simulink model "LoadFlow116BusNetwork_original"  (R2024a)
settings: Solver=FixedStepDiscrete  StartTime=0.0  StopTime=4.5  FixedStep=75e-6  RelTol=1e-3  EnableMultiTasking=on
undefined symbols (not defined in the file or in its folder): D1, D11, Delta
libraries: spsSeriesRLCBranchLib x164, spsLoadFlowBusLib x116, spsDistributedParametersLineLib x79, spsThreePhaseSeriesRLCLoadLib x60, spsThreePhaseTransformerTwoWindingsLib x52, spsThreePhaseParallelRLCLoadLib x44, spsThreePhaseVIMeasurementLib x44, spsSynchronousMachinepuStandardLib x28, spsExcitationSystemLib x28, spsHydraulicTurbineandGovernorLib x28, spsGenericPowerSystemStabilizerLib x28, spsMultiBandPowerSystemStabilizerLib x28
(part 1 of 15)
settings Model: Creator=The MathWorks, Inc.  LastModifiedBy=dilu2
settings SolverCC: AlgebraicLoopSolver=TrustRegion
settings DataIOCC: SaveFormat=StructureWithTime  SaveOutput=off  SignalLogging=off  DSMLogging=off  SaveTime=off  ReturnWorkspaceOutputs=off
settings OptimizationCC: ExpressionDepthLimit=2147483647  LifeSpan=inf
settings DebuggingCC: UnderspecifiedInitializationDetection=Classic  MergeDetectMultiDrivingBlocksExec=none  SolverPrmCheckMsg=warning  FcnCallInpInsideContextMsg=warning  UnconnectedInputMsg=warning  UnconnectedOutputMsg=warning  UnconnectedLineMsg=warning  StateNameClashWarn=warning  SFUnexpectedBacktrackingDiag=warning  SFNoUnconditionalDefaultTransitionDiag=warning  SFExecutionAtInitializationDiag=none  ArithmeticOperatorsInVariantConditions=warning
settings HardwareCC: ProdBitPerPointer=32  ProdBitPerSizeT=32  ProdBitPerPtrDiffT=32  ProdLargestAtomicFloat=None  ProdIntDivRoundTo=Undefined  ProdEndianess=Unspecified  ProdWordSize=32  ProdHWDeviceType=32-bit Generic
settings ModelReferenceCC: EnableRefExpFcnMdlSchedulingChecks=on  PropagateSignalLabelsOutOfModel=off
settings SFSimCC: SimUseLocalCustomCode=off  CustomCodeUndefinedFunction=UseInterfaceOnly
settings RTWCC: RTWUseLocalCustomCode=off  GPUComputeCapability=3.5
settings CodeAppCC: StateflowObjectComments=on
settings GRTTargetCC: TargetLangStandard=C89/C90 (ANSI)  CombineOutputUpdateFcns=off  GRTInterface=on
settings ConfigComp: CovMetricSettings=dw  CovSaveCumulativeToWorkspaceVar=on  CovSaveSingleToWorkspaceVar=on  CovExternalEMLEnable=off  CovSFcnEnable=off
settings SimscapeCC: SimscapeNormalizeSystem=off

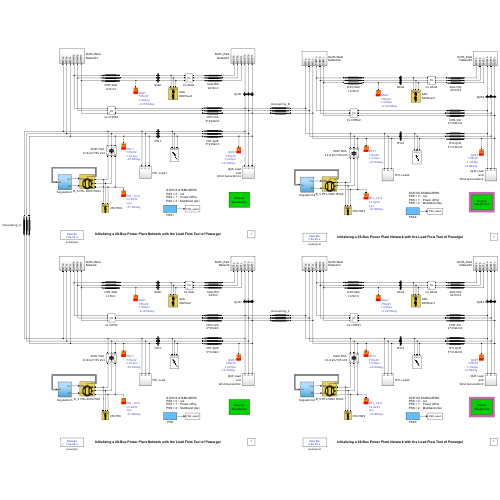
[thumbnail: Simulink's stored preview of the top-level diagram]
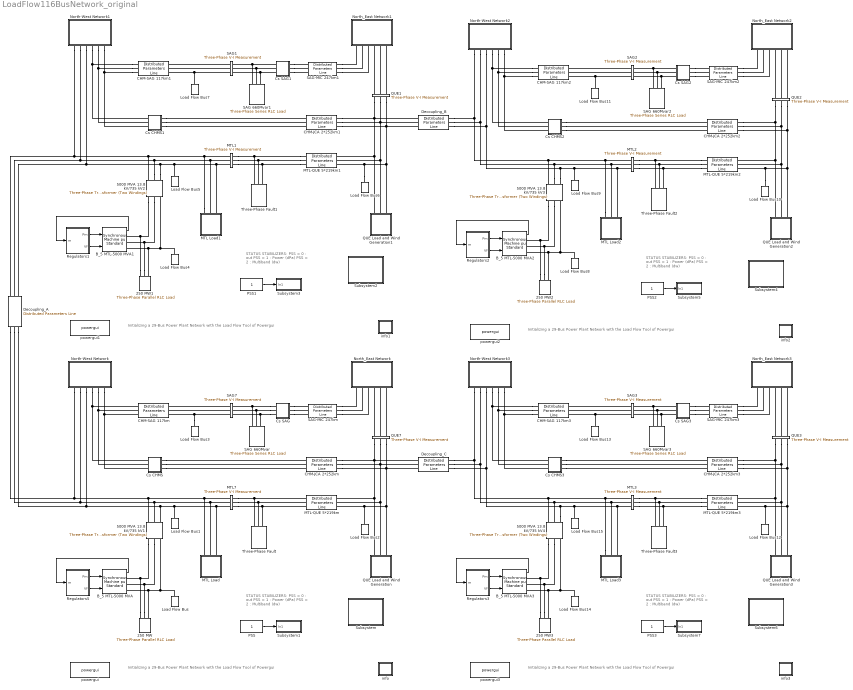
== system LoadFlow116BusNetwork_original ==
  note: Initializing a 29-Bus Power Plant Network with the Load Flow Tool of Powergui
  note: STATUS STABILIZERS:
      | PSS = 0 :  out
      | PSS = 1 :  Power (dPa)
      | PSS = 2 :  Multiband (dw)
  note: STATUS STABILIZERS:
      | PSS = 0 :  out
      | PSS = 1 :  Power (dPa)
      | PSS = 2 :  Multiband (dw)
  note: Initializing a 29-Bus Power Plant Network with the Load Flow Tool of Powergui
  note: Initializing a 29-Bus Power Plant Network with the Load Flow Tool of Powergui
  note: STATUS STABILIZERS:
      | PSS = 0 :  out
      | PSS = 1 :  Power (dPa)
      | PSS = 2 :  Multiband (dw)
  note: STATUS STABILIZERS:
      | PSS = 0 :  out
      | PSS = 1 :  Power (dPa)
      | PSS = 2 :  Multiband (dw)
  note: Initializing a 29-Bus Power Plant Network with the Load Flow Tool of Powergui
  250 MW{,1..3} (4 alike) : spsThreePhaseParallelRLCLoadLib/Three-Phase Parallel RLC Load  LConnTagsString=A|B|C  Configuration=Y (grounded)  NominalVoltage=(13800)*1  Vabc=[1e3 1e3 1e3]  Vabcp=[1e3 1e3 1e3]  NominalFrequency=60  UnbalancedPower=off  ActivePower=250000000  InductivePower=0  CapacitivePower=0  Pabc=[10e3 9e3 11e3]  QLabc=[100 90 110]  QCabc=[100 90 110]  Pabcp=[10e3 9e3 11e3]  QLabcp=[100 90 110]  QCabcp=[100 90 110]  Measurements=None  LoadType=constant PQ
  5000 MVA 13.8 kV/735 kV{1..4} (4 alike) : spsThreePhaseTransformerTwoWindingsLib/Three-Phase Transformer (Two Windings)  Winding1Connection=Delta (D1)  Winding2Connection=Yg  CoreType=Three single-phase transformers  SetSaturation=off  Hysteresis=off  DataFile='basic_model'  SetInitialFlux=off  Measurements=None  UNITS=pu  NominalPower=[ 5000e6 60 ]  Winding1="[ 13.8e3 0.002  0.0]"  Winding2=[ 735e3 0.002 0.12]  Rm=500  Lm=500  L0=0.5  Saturation="[ 0,0  ;  0.005,1.2  ;  1.0,1.4 ]"  InitialFluxes=[ 0.8 , -0.8 , 0.7 ]  BreakLoop=off  DiscreteSolver=Trapezoidal iterative  DataType=off  TransfoNumber=0
  B_5 MTL-5000 MVA{,1..3} (4 alike) : spsSynchronousMachinepuStandardLib/Synchronous Machine pu Standard  PresetModel=No  MechanicalLoad=Mechanical power Pm  ShowDetailedParameters=on  RotorType=Salient-pole  Units=per unit standard parameters  MeasurementBus=off  NominalParameters="[5000E6  13800   60 ]"  Reactances1=[ 31 32 33 34 35 36 37 ]  Reactances2=[ 1.305, 0.296, 0.252, 0.474, 0.243, 0.18 ]  dAxisTimeConstants=Short-circuit  qAxisTimeConstants=Open-circuit  TimeConstants1=[]  TimeConstants2=[]  TimeConstants3=[]  TimeConstants4=[]  TimeConstants5=[ 1.01, 0.053, 0.1 ]  TimeConstants6=[]  TimeConstants7=[]  TimeConstants8=[]  StatorResistance=2.8544e-3  Mechanical="[ 3.7 0  32]"  PolePairs=32  InitialConditions=[0 -113.876 0.904539 0.904539 0.904539 -42.1129 -162.113 77.8871 1.28555]  SetSaturation=off  Saturation=[0.6404,0.7127,0.8441,0.9214,0.9956,1.082,1.19,1.316,1.457;0.7,0.7698,0.8872,0.9466,0.9969,1.046,1.1,1.151,1.201]  LoadFlowParameters=[1 4000000000 0 0 0]  TsPowergui=0  TsBlock=-1  IterativeModel=Trapezoidal non iterative  IterativeDiscreteModel=Trapezoidal non iterative  BusType=PV  Pref=4500000000  Qref=0  Qmin=-Inf  Qmax=Inf  PLF=0  QLF=0
  CHM-JCA 2*252km : spsDistributedParametersLineLib/Distributed Parameters Line  Phases=3  Length=252  Frequency=60  Resistance="[0.01273  0.3864]/2"  Inductance="[0.9337e-3  4.1264e-3]/2"  Capacitance=[12.74e-9 7.751e-9]*2  x1=[-0.0015 2.79983584355551e-08 40957.0521348616 -638802.206166497;-0.001425 2.7893105015594e-08 58999.9677158828 -637388.990068573;-0.00135 2.77655542742622e-08 76995.7196254415 -635466.254964366;-0.001275 2.76158081736708e-08 94929.9223348058 -633035.537858901;-0.0012 2.74439864185614e-08 112788.239516732 -630098.78183024;-0.001125 2.72502263606161e-08 130556.395505707 -626658.334476219;-0.00105 2.70346828886605e-08 148220.186709694 -622716.946037811;-0.000975 2.67975283048483e-08 165765.49296427 -618277.767200629;-0.0009 2.65389521869251e-08 183178.288820068 -613344.346576314;-0.000825 2.62591612366833e-08 200444.654754505 -607920.62786583;-0.00075 2.59583791147275e-08 217550.788298837 -602010.946706926;-0.000675 2.56368462616839e-08 234483.015071642 -595620.027208302;-0.0006 2.52948197059956e-08 251227.799709909 -588752.978173219;-0.000525 2.49325728584581e-08 267771.756689002 -581415.289015608;-0.00045 2.45503952936587e-08 284101.661022843 -573612.825371909;-0.000375 2.41485925184951e-08 300204.458835764 -565351.824412179;-0.0003 2.37274857279582e-08 316067.277797573 -556638.889854187;-0.000225 2.3287411548373e-08 331677.437413503 -547480.986684506;-0.00015 2.28287217683054e-08 347022.459160799 -537885.435590809;-7.5e-05 2.23517830573473e-08 362090.076463864 -527859.907109824]  x2=[-0.0015 1.96439398291852e-08 -210407.400599635 -626129.029139422;-0.001425 1.95042039382265e-08 -192622.277099833 -631827.111409279;-0.00135 1.93488766850639e-08 -174683.174298938 -637020.120753555;-0.001275 1.91780822359271e-08 -156604.43244125 -641703.905960035;-0.0012 1.89919571212853e-08 -138400.503396396 -645874.72288249;-0.001125 1.87906501267075e-08 -120085.939106726 -649529.237433687;-0.00105 1.85743221739249e-08 -101675.379954711 -652664.52825061;-0.000975 1.83431461921932e-08 -83183.5430596452 -655278.089029752;-0.0009 1.8097306980055e-08 -64625.2105130086 -657367.830530614;-0.000825 1.7837001057615e-08 -46015.2175618868 -658932.082245816;-0.00075 1.75624365094449e-08 -27368.4407499025 -659969.593736469;-0.000675 1.72738328182434e-08 -8699.7860251338 -660479.535631762;-0.0006 1.69714206893854e-08 9975.82317547212 -660461.500291947;-0.000525 1.66554418664999e-08 28643.4578556668 -659915.502134199;-0.00045 1.6326148938223e-08 47288.1953939113 -658841.97762109;-0.000375 1.59838051362834e-08 65895.1314722915 -657241.784911691;-0.0003 1.56286841250783e-08 84449.3919908021 -655116.203175571;-0.000225 1.52610697829104e-08 102936.144957474 -652466.931570246;-0.00015 1.48812559750603e-08 121340.612344843 -649296.087882902;-7.5e-05 1.44895463188746e-08 139648.081903277 -645606.206837468]  x3=[-0.0015 6.74615242643494e-11 -389.356346677576 1012.15852814398;-0.001425 6.66063511630319e-11 -417.814729884147 1000.74710827411;-0.00135 6.56979339637061e-11 -445.939118388429 988.535706477818;-0.001275 6.47369988411817e-11 -473.707029984568 975.534084362876;-0.0012 6.37243139522931e-11 -501.096267428898 961.752635227066;-0.001125 6.26606888218456e-11 -528.084936184076 947.202375749965;-0.00105 6.15469736954946e-11 -554.651461921238 931.894937186371;-0.000975 6.03840588600718e-11 -580.774607766193 915.842556068461;-0.0009 5.91728739319033e-11 -606.433491275848 899.058064424092;-0.000825 5.7914387113689e-11 -631.607601131322 881.554879519071;-0.00075 5.66096044205358e-11 -656.276813534371 863.346993131604;-0.000675 5.52595688757648e-11 -680.421408294053 844.44896036748;-0.0006 5.38653596771343e-11 -704.022084590741 824.875888024941;-0.000525 5.24280913341456e-11 -727.059976404907 804.643422518539;-0.00045 5.0948912777121e-11 -749.516667598325 783.767737371633;-0.000375 4.94290064387669e-11 -771.374206635655 762.26552028752;-0.0003 4.78695873089548e-11 -792.615120934621 740.153959809543;-0.000225 4.62719019634771e-11 -813.22243083333 717.45073158083;-0.00015 4.46372275675538e-11 -833.179663163552 694.173984214655;-7.5e-05 4.29668708548854e-11 -852.470864419117 670.342324786718]  x4=[-0.0015 5.35912228760876e-11 -2387.01909458833 -10068.0123244672;-0.001425 5.47734177538654e-11 -2101.43699245865 -10131.4710131204;-0.00135 5.59118275995522e-11 -1814.17503375026 -10186.8307588624;-0.001275 5.70055423857356e-11 -1525.4628512777 -10234.0473079595;-0.0012 5.80536878135499e-11 -1235.5312371422 -10273.0829162248;-0.001125 5.90554260115772e-11 -944.611958239979 -10303.9063791903;-0.00105 6.00099562056291e-11 -652.937570991393 -10326.4930570513;-0.000975 6.09165153588735e-11 -360.741235438837 -10340.8248943632;-0.0009 6.17743787817938e-11 -68.2565288621972 -10346.8904344744;-0.000825 6.25828607114957e-11 224.282740939255 -10344.6848286851;-0.00075 6.33413148598947e-11 516.642722549241 -10334.2098401227;-0.000675 6.40491349303493e-11 808.589707871721 -10315.4738423328;-0.0006 6.47057551023253e-11 1099.89031895356 -10288.4918125854;-0.000525 6.53106504837036e-11 1390.31169454332 -10253.2853199022;-0.00045 6.58633375303718e-11 1679.62167623695 -10209.8825078148;-0.000375 6.63633744327611e-11 1967.58899406166 -10158.3180718671;-0.0003 6.68103614690224e-11 2253.98345134964 -10098.6332318802;-0.000225 6.72039413245583e-11 2538.57610875372 -10030.875699002;-0.00015 6.75437993776541e-11 2821.13946725797 -9955.09963756763;-7.5e-05 6.78296639509821e-11 3101.44765003698 -9871.36562180108]  x5=0.00142516474882927  V1=ones(3,3)  V2=ones(3,3)  I1=ones(3,3)  I2=ones(3,3)  nHarmo=1  Measurements=None  Decoupling=off  VsMag0=[ 1 1 1]  VrMag0=[ 1 1 1]  VsAngle0=[0 -120 120]  VrAngle0=[0 -120 120]  IsMag0=[ 1 1 1]  IrMag0=[ 1 1 1]  IsAngle0=[0 -120 120]  IrAngle0=[0 -120 120]
      settings: AttributesFormatString=\n  LibrarySourceBlock=sps_lib/Power Grid Elements/Distributed Parameters Line
  CHM-JCA 2*252km1 : spsDistributedParametersLineLib/Distributed Parameters Line  Phases=3  Length=252  Frequency=60  Resistance="[0.01273  0.3864]/2"  Inductance="[0.9337e-3  4.1264e-3]/2"  Capacitance=[12.74e-9 7.751e-9]*2  x1=[-0.0015 7.55859688120085e-09 40957.0521347763 -638802.206166561;-0.001425 7.87146395364578e-09 58999.9677157988 -637388.990068633;-0.00135 8.17803869824361e-09 76995.7196253592 -635466.254964424;-0.001275 8.47807604383424e-09 94929.922334725 -633035.537858955;-0.0012 8.77133614515435e-09 112788.239516653 -630098.781830291;-0.001125 9.05758457456597e-09 130556.395505629 -626658.334476266;-0.00105 9.33659250945436e-09 148220.186709618 -622716.946037854;-0.000975 9.60813691514536e-09 165765.492964196 -618277.767200669;-0.0009 9.87200072319581e-09 183178.288819996 -613344.346576351;-0.000825 1.01279730049148e-08 200444.654754435 -607920.627865863;-0.00075 1.03758491399769e-08 217550.788298769 -602010.946706956;-0.000675 1.06154309799923e-08 234483.015071576 -595620.027208328;-0.0006 1.08465270069038e-08 251227.799709845 -588752.978173242;-0.000525 1.10689524860834e-08 267771.75668894 -581415.289015627;-0.00045 1.12825296140063e-08 284101.661022783 -573612.825371925;-0.000375 1.14870876603843e-08 300204.458835706 -565351.824412191;-0.0003 1.16824631046448e-08 316067.277797518 -556638.889854195;-0.000225 1.18684997666472e-08 331677.43741345 -547480.98668451;-0.00015 1.20450489315303e-08 347022.459160749 -537885.43559081;-7.5e-05 1.2211969468593e-08 362090.076463816 -527859.907109821]  x2=[-0.0015 5.57833938393212e-09 -210407.400599694 -626129.029139484;-0.001425 5.75756020399417e-09 -192622.277099891 -631827.111409339;-0.00135 5.93217851852278e-09 -174683.174298994 -637020.120753612;-0.001275 6.10205474030905e-09 -156604.432441306 -641703.90596009;-0.0012 6.26705307290048e-09 -138400.503396451 -645874.722882543;-0.001125 6.42704161915457e-09 -120085.93910678 -649529.237433737;-0.00105 6.58189248667534e-09 -101675.379954764 -652664.528250658;-0.000975 6.73148189004859e-09 -83183.5430596976 -655278.089029798;-0.0009 6.87569024979407e-09 -64625.21051306 -657367.830530658;-0.000825 7.01440228795544e-09 -46015.2175619372 -658932.082245856;-0.00075 7.14750712025178e-09 -27368.4407499517 -659969.593736507;-0.000675 7.27489834471672e-09 -8699.78602518191 -660479.535631798;-0.0006 7.39647412675457e-09 9975.8231754252 -660461.50029198;-0.000525 7.51213728054534e-09 28643.4578556211 -659915.502134229;-0.00045 7.62179534673359e-09 47288.1953938668 -658841.977621118;-0.000375 7.72536066633905e-09 65895.1314722483 -657241.784911716;-0.0003 7.82275045082982e-09 84449.3919907603 -655116.203175593;-0.000225 7.91388684830229e-09 102936.144957434 -652466.931570265;-0.00015 7.99869700571475e-09 121340.612344804 -649296.087882919;-7.5e-05 8.07711312712502e-09 139648.08190324 -645606.206837482]  x3=[-0.0015 3.15277693640631e-11 -389.356346677657 1012.15852814422;-0.001425 3.20576641633681e-11 -417.814729884204 1000.74710827436;-0.00135 3.25619325564397e-11 -445.939118388461 988.535706478099;-0.001275 3.30401714388399e-11 -473.707029984576 975.534084363178;-0.0012 3.34919985137235e-11 -501.096267428882 961.752635227389;-0.001125 3.39170525974399e-11 -528.084936184035 947.202375750308;-0.00105 3.43149939082583e-11 -554.651461921173 931.894937186735;-0.000975 3.46855043379834e-11 -580.774607766104 915.842556068845;-0.0009 3.50282877062468e-11 -606.433491275735 899.058064424495;-0.000825 3.53430699972685e-11 -631.607601131185 881.554879519494;-0.00075 3.56295995789016e-11 -656.27681353421 863.346993132046;-0.000675 3.58876474037824e-11 -680.421408293868 844.448960367941;-0.0006 3.6117007192428e-11 -704.022084590533 824.87588802542;-0.000525 3.63174955981328e-11 -727.059976404675 804.643422519036;-0.00045 3.64889523535328e-11 -749.51666759807 783.767737372148;-0.000375 3.6631240398721e-11 -771.374206635377 762.265520288052;-0.0003 3.67442459908112e-11 -792.61512093432 740.153959810092;-0.000225 3.68278787948623e-11 -813.222430833007 717.450731581396;-0.00015 3.68820719560901e-11 -833.179663163206 694.173984215237;-7.5e-05 3.69067821533109e-11 -852.470864418749 670.342324787315]  x4=[-0.0015 -1.01395513576639e-11 -2387.01909458939 -10068.0123244686;-0.001425 -9.2349393761498e-12 -2101.43699245972 -10131.4710131218;-0.00135 -8.32294512539771e-12 -1814.17503375135 -10186.8307588638;-0.001275 -7.40429763965771e-12 -1525.4628512788 -10234.0473079608;-0.0012 -6.47973127167411e-12 -1235.53123714331 -10273.0829162261;-0.001125 -5.54998510565516e-12 -944.611958241099 -10303.9063791916;-0.00105 -4.61580236646036e-12 -652.937570992522 -10326.4930570526;-0.000975 -3.67792982547795e-12 -360.741235439974 -10340.8248943645;-0.0009 -2.73711720366728e-12 -68.2565288633418 -10346.8904344757;-0.000825 -1.79411657224329e-12 224.282740938104 -10344.6848286863;-0.00075 -8.49681751482354e-13 516.642722548085 -10334.2098401239;-0.000675 9.54322918701537e-14 808.589707870561 -10315.4738423339;-0.0006 1.0404700481087e-12 1099.8903189524 -10288.4918125865;-0.000525 1.98467606851051e-12 1390.31169454216 -10253.2853199033;-0.00045 2.92729556922973e-12 1679.62167623578 -10209.8825078159;-0.000375 3.86757503466002e-12 1967.58899406049 -10158.3180718681;-0.0003 4.80476281978348e-12 2253.98345134847 -10098.6332318812;-0.000225 5.73810975102415e-12 2538.57610875255 -10030.875699003;-0.00015 6.66686972512587e-12 2821.13946725681 -9955.09963756861;-7.5e-05 7.59030030557586e-12 3101.44765003582 -9871.36562180203]  x5=0.00142516474882927  V1=ones(3,3)  V2=ones(3,3)  I1=ones(3,3)  I2=ones(3,3)  nHarmo=1  Measurements=None  Decoupling=off  VsMag0=[ 1 1 1]  VrMag0=[ 1 1 1]  VsAngle0=[0 -120 120]  VrAngle0=[0 -120 120]  IsMag0=[ 1 1 1]  IrMag0=[ 1 1 1]  IsAngle0=[0 -120 120]  IrAngle0=[0 -120 120]
      settings: AttributesFormatString=\n  LibrarySourceBlock=sps_lib/Power Grid Elements/Distributed Parameters Line
  CHM-JCA 2*252km2 : spsDistributedParametersLineLib/Distributed Parameters Line  Phases=3  Length=252  Frequency=60  Resistance="[0.01273  0.3864]/2"  Inductance="[0.9337e-3  4.1264e-3]/2"  Capacitance=[12.74e-9 7.751e-9]*2  x1=[-0.0015 3.38779287371205e-09 -52695.4931205123 -817990.561269677;-0.001425 3.42285731802461e-09 -29549.3766892988 -819153.330536665;-0.00135 3.45518558256862e-09 -6379.63893848035 -819661.281164688;-0.001275 3.48475182462404e-09 16795.1985980936 -819514.007105786;-0.0012 3.51153240938935e-09 39956.6103098835 -818711.626088589;-0.001125 3.53550592887483e-09 63086.0813187483 -817254.779524204;-0.00105 3.55665321901583e-09 86165.1222794564 -815144.631993486;-0.000975 3.57495737499217e-09 109175.284159785 -812382.870316082;-0.0009 3.59040376474162e-09 132098.172988394 -808971.702202023;-0.000825 3.60298004065655e-09 154915.464558685 -804913.854486906;-0.00075 3.61267614945443e-09 177608.919076895 -800212.570952106;-0.000675 3.61948434021423e-09 200160.395742702 -794871.609731751;-0.0006 3.62339917057243e-09 222551.86725071 -788895.240308519;-0.000525 3.62441751107354e-09 244765.434201194 -782288.240100687;-0.00045 3.62253854767175e-09 266783.339408616 -775055.89064313;-0.000375 3.61776378238165e-09 288587.982096435 -767203.973365345;-0.0003 3.61009703207755e-09 310161.931966912 -758738.764969866;-0.000225 3.59954442544235e-09 331487.94313461 -749667.032414763;-0.00015 3.58611439806833e-09 352548.967912502 -739996.027504238;-7.5e-05 3.56981768571388e-09 373328.170439625 -729733.481091645]  x2=[-0.0015 2.09840834715528e-09 -269861.28631546 -765335.489949649;-0.001425 2.12693418151797e-09 -248116.944399075 -772658.724453982;-0.00135 2.15375977723914e-09 -226174.261593654 -779364.307396061;-0.001275 2.17886369034802e-09 -204050.778544097 -785446.878435482;-0.0012 2.20222585316057e-09 -181764.180424253 -790901.575258022;-0.001125 2.22382759032128e-09 -159332.282799664 -795724.0374625;-0.00105 2.24365163373199e-09 -136773.01738607 -799910.410046417;-0.000975 2.26168213635572e-09 -114104.417715075 -803457.346487582;-0.0009 2.27790468488455e-09 -91344.6047184146 -806362.011419275;-0.000825 2.29230631126139e-09 -68511.7722423618 -808622.082896792;-0.00075 2.30487550304646e-09 -45624.1725038437 -810235.754253574;-0.000675 2.31560221262018e-09 -22700.1014998993 -811201.735545428;-0.0006 2.32447786521504e-09 242.115617860982 -811519.25458169;-0.000525 2.33149536577014e-09 23184.1391921008 -811188.0575425;-0.00045 2.33664910460293e-09 46107.6297201997 -810208.409181705;-0.000375 2.33993496189342e-09 68994.2625145706 -808581.092615214;-0.0003 2.34135031097759e-09 91825.742351135 -806307.408694992;-0.000225 2.34089402044701e-09 114583.818094245 -803389.174969176;-0.00015 2.33856645505338e-09 137250.297286361 -799828.724229156;-7.5e-05 2.33436947541683e-09 159807.060690827 -795628.902644778]  x3=[-0.0015 7.09671795045562e-12 -353.825063947035 -933.331217283161;-0.001425 7.0863399131954e-12 -327.297425888444 -942.960561677136;-0.00135 7.07029716423321e-12 -300.508151275417 -951.836117825887;-0.001275 7.04860252789711e-12 -273.478655044189 -959.950790745628;-0.0012 7.02127334654744e-12 -246.230544160483 -967.298093690987;-0.001125 6.98833146671362e-12 -218.785600347228 -973.872153340407;-0.00105 6.94980322163037e-12 -191.165762672588 -979.66771449119;-0.000975 6.90571941018731e-12 -163.393110012202 -984.680144260428;-0.0009 6.85611527230879e-12 -135.48984339967 -988.905435788455;-0.000825 6.80103046078367e-12 -107.478268279388 -992.340211441873;-0.00075 6.74050900956746e-12 -79.3807766759173 -994.981725513579;-0.000675 6.67459929858224e-12 -51.2198292941379 -996.827866417641;-0.0006 6.60335401504253e-12 -23.0179375645104 -997.877158377266;-0.000525 6.5268301113379e-12 5.20235435221977 -998.128762604516;-0.00045 6.44508875950611e-12 33.4184875864796 -997.582477970823;-0.000375 6.35819530233314e-12 61.6079065930828 -996.238741167764;-0.0003 6.26621920111914e-12 89.748077181788 -994.098626357979;-0.000225 6.16923398015213e-12 117.816504530786 -991.163844316503;-0.00015 6.06731716793383e-12 145.790751168715 -987.436741063195;-7.5e-05 5.96055023520455e-12 173.648454910832 -982.92029598737]  x4=[-0.0015 5.81566752832242e-12 -3930.11452440085 -10267.867125637;-0.001425 6.00314064654812e-12 -3638.26562484153 -10374.8700196274;-0.00135 6.1858149459921e-12 -3343.50835140904 -10473.579401265;-0.001275 6.36354439961439e-12 -3046.07832855782 -10563.9163637803;-0.0012 6.53618693320912e-12 -2746.21331729732 -10645.8086931878;-0.001125 6.70360453897647e-12 -2444.15302512944 -10719.1909260123;-0.00105 6.86566338584394e-12 -2140.13891443007 -10784.0044016197;-0.000975 7.02223392644894e-12 -1834.41400942773 -10840.1973091092;-0.0009 7.17319100069693e-12 -1527.22270193373 -10887.7247287303;-0.000825 7.31841393581245e-12 -1218.81055597909 -10926.5486677911;-0.00075 7.45778664280318e-12 -909.42411151443 -10956.6380910287;-0.000675 7.59119770925961e-12 -599.31068732968 -10977.9689454185;-0.0006 7.71854048841648e-12 -288.71818335124 -10990.5241794019;-0.000525 7.83971318440454e-12 22.1051175254338 -10994.2937565169;-0.00045 7.95461893362462e-12 332.910747909378 -10989.2746634213;-0.000375 8.06316588217891e-12 643.450254535149 -10975.4709123013;-0.0003 8.16526725929756e-12 953.475396872564 -10952.8935376643;-0.000225 8.26084144670191e-12 1262.73834556638 -10921.5605875182;-0.00015 8.34981204384888e-12 1570.9918805473 -10881.497108944;-7.5e-05 8.4321079290044e-12 1877.98958865589 -10832.7351280733]  x5=0.00142516474882927  V1=ones(3,3)  V2=ones(3,3)  I1=ones(3,3)  I2=ones(3,3)  nHarmo=1  Measurements=None  Decoupling=off  VsMag0=[ 1 1 1]  VrMag0=[ 1 1 1]  VsAngle0=[0 -120 120]  VrAngle0=[0 -120 120]  IsMag0=[ 1 1 1]  IrMag0=[ 1 1 1]  IsAngle0=[0 -120 120]  IrAngle0=[0 -120 120]
      settings: AttributesFormatString=\n  LibrarySourceBlock=sps_lib/Power Grid Elements/Distributed Parameters Line
  CHM-JCA 2*252km3 : spsDistributedParametersLineLib/Distributed Parameters Line  Phases=3  Length=252  Frequency=60  Resistance="[0.01273  0.3864]/2"  Inductance="[0.9337e-3  4.1264e-3]/2"  Capacitance=[12.74e-9 7.751e-9]*2  x1=[-0.0015 1.20512797034984e-08 -52695.4931206192 -817990.56126955;-0.001425 1.1991769673533e-08 -29549.3766894013 -819153.330536534;-0.00135 1.19226736063707e-08 -6379.63893857854 -819661.281164554;-0.001275 1.18440467363506e-08 16795.1985979998 -819514.007105648;-0.0012 1.17559519165894e-08 39956.6103097942 -818711.626088447;-0.001125 1.16584595687382e-08 63086.0813186635 -817254.77952406;-0.00105 1.15516476266881e-08 86165.1222793762 -815144.631993337;-0.000975 1.14356014742714e-08 109175.284159709 -812382.870315931;-0.0009 1.13104138770068e-08 132098.172988323 -808971.702201868;-0.000825 1.1176184907944e-08 154915.46455862 -804913.854486748;-0.00075 1.10330218676671e-08 177608.919076834 -800212.570951946;-0.000675 1.08810391985202e-08 200160.395742646 -794871.609731588;-0.0006 1.07203583931234e-08 222551.867250658 -788895.240308353;-0.000525 1.05511078972542e-08 244765.434201148 -782288.240100519;-0.00045 1.03734230071692e-08 266783.339408574 -775055.890642959;-0.000375 1.0187445761451e-08 288587.982096399 -767203.973365172;-0.0003 9.99332482746425e-09 310161.93196688 -758738.764969692;-0.000225 9.79121538251343e-09 331487.943134584 -749667.032414587;-0.00015 9.58127898979644e-09 352548.967912481 -739996.02750406;-7.5e-05 9.36368346925349e-09 373328.17043961 -729733.481091465]  x2=[-0.0015 7.36275622166878e-09 -269861.286315555 -765335.48994954;-0.001425 7.30821921463715e-09 -248116.944399166 -772658.72445387;-0.00135 7.24784012898485e-09 -226174.261593741 -779364.307395945;-0.001275 7.1816672308291e-09 -204050.778544181 -785446.878435363;-0.0012 7.10975341777223e-09 -181764.180424333 -790901.575257899;-0.001125 7.03215617661606e-09 -159332.28279974 -795724.037462375;-0.00105 6.94893753740791e-09 -136773.017386142 -799910.410046289;-0.000975 6.86016402385466e-09 -114104.417715143 -803457.346487451;-0.0009 6.76590660014477e-09 -91344.6047184784 -806362.011419141;-0.000825 6.66624061422056e-09 -68511.7722424214 -808622.082896655;-0.00075 6.56124573754625e-09 -45624.1725038991 -810235.754253435;-0.000675 6.45100590141978e-09 -22700.1014999503 -811201.735545287;-0.0006 6.3356092298794e-09 242.115617814212 -811519.254581546;-0.000525 6.21514796925874e-09 23184.1391920584 -811188.057542354;-0.00045 6.0897184144464e-09 46107.6297201617 -810208.409181557;-0.000375 5.95942083190936e-09 68994.262514537 -808581.092615064;-0.0003 5.8243593795415e-09 91825.7423511058 -806307.40869484;-0.000225 5.68464202340132e-09 114583.81809422 -803389.174969022;-0.00015 5.54038045140557e-09 137250.297286341 -799828.724229001;-7.5e-05 5.39168998404763e-09 159807.060690812 -795628.902644621]  x3=[-0.0015 2.52783376140647e-11 -353.825063947547 -933.331217282041;-0.001425 2.47986248194378e-11 -327.297425888922 -942.960561675995;-0.00135 2.4299088383562e-11 -300.508151275861 -951.836117824726;-0.001275 2.37801276282208e-11 -273.478655044598 -959.950790744448;-0.0012 2.32421574027018e-11 -246.230544160856 -967.298093689789;-0.001125 2.26856077521721e-11 -218.785600347566 -973.872153339192;-0.00105 2.21109235739067e-11 -191.16576267289 -979.667714489959;-0.000975 2.15185642616447e-11 -163.393110012467 -984.680144259181;-0.0009 2.09090033383571e-11 -135.489843399899 -988.905435787194;-0.000825 2.02827280777193e-11 -107.478268279581 -992.340211440599;-0.00075 1.96402391145923e-11 -79.3807766760731 -994.981725512293;-0.000675 1.89820500448228e-11 -51.2198292942568 -996.827866416343;-0.0006 1.83086870146827e-11 -23.0179375645924 -997.877158375958;-0.000525 1.76206883002752e-11 5.20235435217475 -998.1287626032;-0.00045 1.69186038772461e-11 33.4184875864716 -997.582477969499;-0.000375 1.62029949811409e-11 61.6079065931117 -996.238741166432;-0.0003 1.54744336587619e-11 89.748077181854 -994.098626356642;-0.000225 1.47335023108828e-11 117.816504530889 -991.16384431516;-0.00015 1.39807932266865e-11 145.790751168854 -987.436741061849;-7.5e-05 1.32169081102982e-11 173.648454911009 -982.920295986022]  x4=[-0.0015 2.45266682732932e-11 -3930.11452440215 -10267.8671256367;-0.001425 2.50850869107939e-11 -3638.26562484281 -10374.8700196271;-0.00135 2.56234529136328e-11 -3343.5083514103 -10473.5794012646;-0.001275 2.61413359202646e-11 -3046.07832855907 -10563.9163637799;-0.0012 2.66383219429375e-11 -2746.21331729854 -10645.8086931874;-0.001125 2.71140136986292e-11 -2444.15302513065 -10719.1909260118;-0.00105 2.75680309266285e-11 -2140.13891443125 -10784.0044016191;-0.000975 2.80000106925102e-11 -1834.41400942889 -10840.1973091086;-0.0009 2.84096076782587e-11 -1527.22270193486 -10887.7247287297;-0.000825 2.87964944583109e-11 -1218.8105559802 -10926.5486677905;-0.00075 2.91603617612942e-11 -909.424111515516 -10956.638091028;-0.000675 2.9500918717254e-11 -599.310687330739 -10977.9689454178;-0.0006 2.98178930901704e-11 -288.718183352272 -10990.5241794011;-0.000525 3.01110314955797e-11 22.1051175244306 -10994.2937565161;-0.00045 3.03800996031255e-11 332.910747908404 -10989.2746634205;-0.000375 3.06248823238798e-11 643.450254534205 -10975.4709123004;-0.0003 3.08451839822808e-11 953.47539687165 -10952.8935376634;-0.000225 3.10408284725534e-11 1262.7383455655 -10921.5605875173;-0.00015 3.12116593994858e-11 1570.99188054645 -10881.497108943;-7.5e-05 3.13575402034485e-11 1877.98958865507 -10832.7351280723]  x5=0.00142516474882927  V1=ones(3,3)  V2=ones(3,3)  I1=ones(3,3)  I2=ones(3,3)  nHarmo=1  Measurements=None  Decoupling=off  VsMag0=[ 1 1 1]  VrMag0=[ 1 1 1]  VsAngle0=[0 -120 120]  VrAngle0=[0 -120 120]  IsMag0=[ 1 1 1]  IrMag0=[ 1 1 1]  IsAngle0=[0 -120 120]  IrAngle0=[0 -120 120]
      settings: AttributesFormatString=\n  LibrarySourceBlock=sps_lib/Power Grid Elements/Distributed Parameters Line
  CHM-SAG 117km : spsDistributedParametersLineLib/Distributed Parameters Line  Phases=3  Length=117  Frequency=60  Resistance="[0.01273  0.3864]"  Inductance="[0.9337e-3  4.1264e-3]"  Capacitance=[12.74e-9 7.751e-9]  x1=[-0.000675 2.51067295491762e-08 148076.925129456 -635412.044036454;-0.0006 2.47669678355952e-08 165981.19222809 -630971.847683723;-0.000525 2.44074077868738e-08 183752.776501255 -626027.262090147;-0.00045 2.40283368298134e-08 201377.471616397 -620582.239881795;-0.000375 2.36300579879372e-08 218841.188661906 -614641.133726107;-0.0003 2.32128896392574e-08 236129.967409582 -608208.692852444;-0.000225 2.27771652617691e-08 253229.987474221 -601290.05925562;-0.00015 2.23232331668729e-08 270127.579361421 -593890.763585473;-7.5e-05 2.185145622094e-08 286809.23539477 -586016.720725749]  x2=[-0.000675 1.74032777665883e-08 194552.652189026 -614840.258036848;-0.0006 1.71357721344792e-08 211856.770310051 -609094.40535433;-0.000525 1.68545684283118e-08 228991.533370407 -602861.651923628;-0.00045 1.65598914380264e-08 245943.244102674 -596146.98011247;-0.000375 1.62519767239002e-08 262698.351568664 -588955.757526766;-0.0003 1.59310704282446e-08 279243.461991829 -581293.73271982;-0.000225 1.55974290786421e-08 295565.349464046 -573167.03059703;-0.00015 1.52513193828829e-08 311650.966518203 -564582.14751973;-7.5e-05 1.4893018015762e-08 327487.454558145 -555545.9461121]  x3=[-0.000675 1.36248972760017e-11 906.35946632907 -3489.31280860133;-0.0006 1.22128582371722e-11 1004.64242810611 -3462.29477190377;-0.000525 1.07910564263309e-11 1102.12229409766 -3432.50902974044;-0.00045 9.36062841009112e-12 1198.72114039035 -3399.97939237789;-0.000375 7.92271765072273e-12 1294.36174734446 -3364.7318635105;-0.0003 6.47847359208599e-12 1388.96766132214 -3326.79461947354;-0.000225 5.02905074078372e-12 1482.46325580328 -3286.19798671943;-0.00015 3.57560774326631e-12 1574.77379184018 -3242.97441757527;-7.5e-05 2.11930645962757e-12 1665.82547780273 -3197.15846430086]  x4=[-0.000675 4.82056153235792e-11 3.0549351155492 -1206.09020238117;-0.0006 4.89255674784095e-11 37.1501564669208 -1205.52186302311;-0.000525 4.96064092831838e-11 71.2156805516292 -1203.98984793286;-0.00045 5.02475964833807e-11 105.224275910941 -1201.49538177984;-0.000375 5.08486165237627e-11 139.148756594075 -1198.04045860211;-0.0003 5.14089889581056e-11 172.962003890235 -1193.62784021242;-0.000225 5.19282658332593e-11 206.636988006893 -1188.26105399037;-0.00015 5.24060320472349e-11 240.14678967699 -1181.94439006277;-7.5e-05 5.28419056810312e-11 273.464621677788 -1174.68289787411]  x5=0.000661683633385019  V1=ones(3,3)  V2=ones(3,3)  I1=ones(3,3)  I2=ones(3,3)  nHarmo=1  Measurements=None  Decoupling=off  VsMag0=[ 1 1 1]  VrMag0=[ 1 1 1]  VsAngle0=[0 -120 120]  VrAngle0=[0 -120 120]  IsMag0=[ 1 1 1]  IrMag0=[ 1 1 1]  IsAngle0=[0 -120 120]  IrAngle0=[0 -120 120]
      settings: AttributesFormatString=\n  LibrarySourceBlock=sps_lib/Power Grid Elements/Distributed Parameters Line
  CHM-SAG 117km1 : spsDistributedParametersLineLib/Distributed Parameters Line  Phases=3  Length=117  Frequency=60  Resistance="[0.01273  0.3864]"  Inductance="[0.9337e-3  4.1264e-3]"  Capacitance=[12.74e-9 7.751e-9]  x1=[-0.000675 1.00014597526922e-08 148076.925129396 -635412.044036485;-0.0006 1.02112832191752e-08 165981.192228032 -630971.847683751;-0.000525 1.04129439420907e-08 183752.776501199 -626027.262090172;-0.00045 1.06062807169423e-08 201377.471616342 -620582.239881816;-0.000375 1.07911389932703e-08 218841.188661854 -614641.133726125;-0.0003 1.0967370998197e-08 236129.967409532 -608208.692852459;-0.000225 1.11348358545541e-08 253229.987474172 -601290.059255631;-0.00015 1.12933996934979e-08 270127.579361374 -593890.76358548;-7.5e-05 1.14429357615214e-08 286809.235394726 -586016.720725753]  x2=[-0.000675 6.76928505877694e-09 194552.652188964 -614840.258036884;-0.0006 6.89372115213374e-09 211856.77030999 -609094.405354362;-0.000525 7.01264651027898e-09 228991.533370347 -602861.651923657;-0.00045 7.125966066101e-09 245943.244102616 -596146.980112496;-0.000375 7.23358923368072e-09 262698.351568608 -588955.757526789;-0.0003 7.33542998070466e-09 279243.461991775 -581293.732719839;-0.000225 7.43140689723787e-09 295565.349463994 -573167.030597046;-0.00015 7.52144326080176e-09 311650.966518153 -564582.147519743;-7.5e-05 7.60546709770491e-09 327487.454558097 -555545.946112109]  x3=[-0.000675 2.54210404130717e-11 906.359466328927 -3489.31280860151;-0.0006 2.50987695315334e-11 1004.64242810597 -3462.29477190395;-0.000525 2.47564350776556e-11 1102.12229409753 -3432.50902974061;-0.00045 2.43943107083629e-11 1198.72114039022 -3399.97939237805;-0.000375 2.40126859003354e-11 1294.36174734434 -3364.73186351065;-0.0003 2.36118657186056e-11 1388.96766132202 -3326.79461947368;-0.000225 2.3192170572694e-11 1482.46325580316 -3286.19798671957;-0.00015 2.27539359604787e-11 1574.77379184007 -3242.97441757539;-7.5e-05 2.22975122000035e-11 1665.82547780262 -3197.15846430097]  x4=[-0.000675 -3.24287760924174e-12 3.05493511520535 -1206.09020238129;-0.0006 -2.48064505493916e-12 37.1501564665847 -1205.52186302322;-0.000525 -1.71642951093481e-12 71.2156805513011 -1203.98984793296;-0.00045 -9.50841879441663e-13 105.224275910621 -1201.49538177992;-0.000375 -1.84494159498463e-13 139.148756593764 -1198.04045860218;-0.0003 5.82001042252985e-13 172.962003889933 -1193.62784021247;-0.000225 1.34803100127617e-12 206.6369880066 -1188.26105399041;-0.00015 2.1129833649425e-12 240.146789676706 -1181.94439006279;-7.5e-05 2.87624664203663e-12 273.464621677514 -1174.68289787411]  x5=0.000661683633385019  V1=ones(3,3)  V2=ones(3,3)  I1=ones(3,3)  I2=ones(3,3)  nHarmo=1  Measurements=None  Decoupling=off  VsMag0=[ 1 1 1]  VrMag0=[ 1 1 1]  VsAngle0=[0 -120 120]  VrAngle0=[0 -120 120]  IsMag0=[ 1 1 1]  IrMag0=[ 1 1 1]  IsAngle0=[0 -120 120]  IrAngle0=[0 -120 120]
      settings: AttributesFormatString=\n  LibrarySourceBlock=sps_lib/Power Grid Elements/Distributed Parameters Line
  CHM-SAG 117km2 : spsDistributedParametersLineLib/Distributed Parameters Line  Phases=3  Length=117  Frequency=60  Resistance="[0.01273  0.3864]"  Inductance="[0.9337e-3  4.1264e-3]"  Capacitance=[12.74e-9 7.751e-9]  x1=[-0.000675 2.61786173370322e-09 120099.384212667 -820048.654169185;-0.0006 2.6199125353962e-09 143234.62761723 -816325.600271001;-0.000525 2.61986901909439e-09 166255.371452038 -811949.988178161;-0.00045 2.61773121958406e-09 189143.2132867 -806925.315688023;-0.000375 2.61350084578942e-09 211879.856930649 -801255.599446895;-0.0003 2.60718127940656e-09 234447.127058838 -794945.371739191;-0.000225 2.59877757220015e-09 256826.983740818 -787999.67686439;-0.00015 2.58829644196516e-09 279001.53686158 -780424.067104704;-7.5e-05 2.57574626715673e-09 300953.060422641 -772224.598286663]  x2=[-0.000675 2.69389638303589e-09 166130.546631759 -803426.09827287;-0.0006 2.70072670390528e-09 188777.466023468 -798408.377649353;-0.000525 2.70539810517008e-09 211273.47959723 -792752.421584801;-0.00045 2.70790685258358e-09 233600.604383995 -786462.751363953;-0.000375 2.70825094069149e-09 255740.992421824 -779544.394852949;-0.0003 2.70643009443504e-09 277676.945023279 -772002.882480128;-0.000225 2.70244576937087e-09 299390.926923483 -763844.242815092;-0.00015 2.69630115050747e-09 320865.580297539 -755074.99774956;-7.5e-05 2.68800114975915e-09 342083.738636113 -745702.157283861]  x3=[-0.000675 3.88508588795955e-12 655.342290944776 -4153.32595111545;-0.0006 3.85736806398909e-12 772.497655200545 -4133.13889809567;-0.000525 3.82656671900798e-12 889.035496650358 -4109.64787707989;-0.00045 3.79270647514013e-12 1004.86265672685 -4082.8716664309;-0.000375 3.75581439974641e-12 1119.88654497047 -4052.8316706418;-0.0003 3.71591998378741e-12 1234.01521304487 -4019.55190322559;-0.000225 3.67305511824886e-12 1347.15742823904 -3983.05896751914;-0.00015 3.62725406864841e-12 1459.22274639727 -3943.38203541691;-7.5e-05 3.57855344764433e-12 1570.12158421888 -3900.55282405133]  x4=[-0.000675 3.20269812810429e-12 -58.1790322604634 -1899.19040567976;-0.0006 3.23704231372482e-12 -4.46495442907224 -1900.07615984023;-0.000525 3.26879885724817e-12 49.2526926185736 -1899.44302219067;-0.00045 3.29794237297934e-12 102.930967817332 -1897.29149885163;-0.000375 3.32444956403775e-12 156.526961575313 -1893.62330971793;-0.0003 3.34829924098046e-12 209.997830075154 -1888.44138708385;-0.000225 3.36947233874062e-12 263.300829522707 -1881.74987329907;-0.00015 3.38795193186785e-12 316.393350315778 -1873.5541174573;-7.5e-05 3.40372324805815e-12 369.232951105587 -1863.86067112038]  x5=0.000661683633385019  V1=ones(3,3)  V2=ones(3,3)  I1=ones(3,3)  I2=ones(3,3)  nHarmo=1  Measurements=None  Decoupling=off  VsMag0=[ 1 1 1]  VrMag0=[ 1 1 1]  VsAngle0=[0 -120 120]  VrAngle0=[0 -120 120]  IsMag0=[ 1 1 1]  IrMag0=[ 1 1 1]  IsAngle0=[0 -120 120]  IrAngle0=[0 -120 120]
      settings: AttributesFormatString=\n  LibrarySourceBlock=sps_lib/Power Grid Elements/Distributed Parameters Line
  CHM-SAG 117km3 : spsDistributedParametersLineLib/Distributed Parameters Line  Phases=3  Length=117  Frequency=60  Resistance="[0.01273  0.3864]"  Inductance="[0.9337e-3  4.1264e-3]"  Capacitance=[12.74e-9 7.751e-9]  x1=[-0.000675 1.12460662274108e-08 120099.384212611 -820048.654169028;-0.0006 1.10913243486467e-08 143234.627617178 -816325.600270841;-0.000525 1.09277162349012e-08 166255.371451991 -811949.988177999;-0.00045 1.07553726719972e-08 189143.213286659 -806925.315687858;-0.000375 1.05744314287419e-08 211879.856930612 -801255.599446728;-0.0003 1.03850371467967e-08 234447.127058806 -794945.371739022;-0.000225 1.01873412250528e-08 256826.983740791 -787999.67686422;-0.00015 9.98150169860509e-09 279001.536861558 -780424.067104532;-7.5e-05 9.76768311242163e-09 300953.060422624 -772224.598286489]  x2=[-0.000675 7.09354226825218e-09 166130.546631696 -803426.098272706;-0.0006 6.96688565449627e-09 188777.46602341 -798408.377649187;-0.000525 6.83465981894507e-09 211273.479597177 -792752.421584632;-0.00045 6.69697046090842e-09 233600.604383947 -786462.751363782;-0.000375 6.55392764715239e-09 255740.992421781 -779544.394852775;-0.0003 6.40564572391369e-09 277676.945023242 -772002.882479952;-0.000225 6.25224322549296e-09 299390.926923451 -763844.242814915;-0.00015 6.0938427795003e-09 320865.580297512 -755074.99774938;-7.5e-05 5.93057100882862e-09 342083.738636091 -745702.157283679]  x3=[-0.000675 4.89671668253689e-12 655.342290944364 -4153.32595111508;-0.0006 4.16449725133034e-12 772.497655200146 -4133.13889809528;-0.000525 3.42894878474002e-12 889.035496649973 -4109.64787707949;-0.00045 2.69065926895585e-12 1004.86265672648 -4082.87166643048;-0.000375 1.95021888132056e-12 1119.88654497011 -4052.83167064137;-0.0003 1.20821951855088e-12 1234.01521304453 -4019.55190322514;-0.000225 4.65254323584449e-13 1347.15742823871 -3983.05896751868;-0.00015 -2.78082788569624e-13 1459.22274639695 -3943.38203541644;-7.5e-05 -1.02119760559732e-12 1570.12158421858 -3900.55282405085]  x4=[-0.000675 2.03136090483704e-11 -58.1790322605842 -1899.190405679;-0.0006 2.07341659287888e-11 -4.46495442917063 -1900.07615983947;-0.000525 2.11381482342071e-11 49.2526926184975 -1899.4430221899;-0.00045 2.15252330273515e-11 102.930967817278 -1897.29149885085;-0.000375 2.18951108785609e-11 156.526961575282 -1893.62330971715;-0.0003 2.22474861131405e-11 209.997830075145 -1888.44138708307;-0.000225 2.25820770477192e-11 263.300829522721 -1881.74987329828;-0.00015 2.28986162154232e-11 316.393350315814 -1873.55411745651;-7.5e-05 2.31968505796853e-11 369.232951105646 -1863.86067111959]  x5=0.000661683633385019  V1=ones(3,3)  V2=ones(3,3)  I1=ones(3,3)  I2=ones(3,3)  nHarmo=1  Measurements=None  Decoupling=off  VsMag0=[ 1 1 1]  VrMag0=[ 1 1 1]  VsAngle0=[0 -120 120]  VrAngle0=[0 -120 120]  IsMag0=[ 1 1 1]  IrMag0=[ 1 1 1]  IsAngle0=[0 -120 120]  IrAngle0=[0 -120 120]
      settings: AttributesFormatString=\n  LibrarySourceBlock=sps_lib/Power Grid Elements/Distributed Parameters Line
  Cs CHMS : Subsystem  mask{Xc=33/2}
      mask prompts: Xc "Condensator Reactance at  60Hz  (ohm):"
      mask help: Series Compensation
      mask init:
      | Cs=1/Xc/(2*pi*60);
      mask Display: disp('Cs')
  Cs CHMS1 : Subsystem  mask{Xc=33/2}
      mask prompts: Xc "Condensator Reactance at  60Hz  (ohm):"
      mask help: Series Compensation
      mask init:
      | Cs=1/Xc/(2*pi*60);
      mask Display: disp('Cs')
  Cs CHMS2 : Subsystem  mask{Xc=33/2}
      mask prompts: Xc "Condensator Reactance at  60Hz  (ohm):"
      mask help: Series Compensation
      mask init:
      | Cs=1/Xc/(2*pi*60);
      mask Display: disp('Cs')
  Cs CHMS3 : Subsystem  mask{Xc=33/2}
      mask prompts: Xc "Condensator Reactance at  60Hz  (ohm):"
      mask help: Series Compensation
      mask init:
      | Cs=1/Xc/(2*pi*60);
      mask Display: disp('Cs')
  Cs SAG : Subsystem  mask{Xc=22}
      mask prompts: Xc "Condensator Reactance at  60Hz  (ohm):"
      mask help: Series Compensation
      mask init:
      | Cs=1/Xc/(2*pi*60);
      mask Display: disp('Cs')
  Cs SAG1 : Subsystem  mask{Xc=22}
      mask prompts: Xc "Condensator Reactance at  60Hz  (ohm):"
      mask help: Series Compensation
      mask init:
      | Cs=1/Xc/(2*pi*60);
      mask Display: disp('Cs')
  Cs SAG2 : Subsystem  mask{Xc=22}
      mask prompts: Xc "Condensator Reactance at  60Hz  (ohm):"
      mask help: Series Compensation
      mask init:
      | Cs=1/Xc/(2*pi*60);
      mask Display: disp('Cs')
  Cs SAG3 : Subsystem  mask{Xc=22}
      mask prompts: Xc "Condensator Reactance at  60Hz  (ohm):"
      mask help: Series Compensation
      mask init:
      | Cs=1/Xc/(2*pi*60);
      mask Display: disp('Cs')
  Decoupling_A : spsDistributedParametersLineLib/Distributed Parameters Line  Phases=3  Length=252  Frequency=60  Resistance="[0.01273  0.3864]/2"  Inductance="[0.9337e-3  4.1264e-3]/2"  Capacitance=[12.74e-9 7.751e-9]*2  x1=[-0.0015 2.83450844321183e-08 351989.932817852 531657.75574173;-0.001425 2.96023910382486e-08 366879.510878085 521494.300151841;-0.00135 3.08360339459147e-08 381475.811070767 510913.96999754;-0.001275 3.20450269998515e-08 395767.165336854 499925.22303287;-0.0012 3.322840374951e-08 409742.149386412 488536.843494019;-0.001125 3.43852182216228e-08 423389.591831016 476757.935077344;-0.00105 3.55145456764007e-08 436698.583113988 464597.913662009;-0.000975 3.66154833467557e-08 449658.48423133 452066.499783079;-0.0009 3.7687151159959e-08 462258.935236384 439173.710861072;-0.000825 3.87286924411577e-08 474489.863521409 425929.853194185;-0.00075 3.97392745981878e-08 486341.491869473 412345.513719601;-0.000675 4.07180897871355e-08 497804.346270211 398431.551550447;-0.0006 4.16643555581149e-08 508869.263493203 384199.08929519;-0.000525 4.25773154807472e-08 519527.398412918 369659.504166394;-0.00045 4.3456239748839e-08 529770.231079379 354824.418885948;-0.000375 4.43004257637783e-08 539589.573528871 339705.69239404;-0.0003 4.51091986961814e-08 548977.576329281 324315.410369303;-0.000225 4.58819120253405e-08 557926.734854812 308665.87556771;-0.00015 4.66179480560434e-08 566429.895285065 292769.597987934;-7.5e-05 4.73167184123488e-08 574480.260323696 276639.284871051]  x2=[-0.0015 1.11972632592692e-07 351989.932817863 531657.75574166;-0.001425 1.11637008387708e-07 366879.510878098 521494.300151773;-0.00135 1.11212143266321e-07 381475.811070781 510913.969997476;-0.001275 1.10698376859211e-07 395767.16533687 499925.223032808;-0.0012 1.10096119863381e-07 409742.14938643 488536.843493961;-0.001125 1.09405853713859e-07 423389.591831035 476757.935077289;-0.00105 1.08628130198845e-07 436698.583114008 464597.913661957;-0.000975 1.07763571018615e-07 449658.484231353 452066.49978303;-0.0009 1.06812867288551e-07 462258.935236408 439173.710861026;-0.000825 1.05776778986668e-07 474489.863521434 425929.853194142;-0.00075 1.04656134346103e-07 486341.4918695 412345.513719561;-0.000675 1.03451829193033e-07 497804.346270239 398431.55155041;-0.0006 1.02164826230573e-07 508869.263493232 384199.089295157;-0.000525 1.00796154269199e-07 519527.39841295 369659.504166365;-0.00045 9.9346907404334e-08 529770.231079411 354824.418885922;-0.000375 9.7818244141749e-08 539589.573528904 339705.692394017;-0.0003 9.62113864714665e-08 548977.576329316 324315.410369284;-0.000225 9.45276188909222e-08 557926.734854848 308665.875567694;-0.00015 9.27682873781576e-08 566429.895285103 292769.597987921;-7.5e-05 9.09347983158653e-08 574480.260323735 276639.284871042]  x3=[-0.0015 3.90568306170648e-10 1931.73943952734 4320.02713013127;-0.001425 4.03615139627146e-10 2053.09694959988 4263.68907149061;-0.00135 4.16339329316546e-10 2172.81324538435 4203.94268504283;-0.001275 4.28730703716295e-10 2290.79262750561 4140.8357311351;-0.0012 4.40779357351293e-10 2406.94078505075 4074.41865650081;-0.001125 4.52475658712175e-10 2521.16487095974 4004.74455393322;-0.00105 4.63810257954592e-10 2633.37357624601 3931.86911984386;-0.000975 4.74774094373335e-10 2743.47720298739 3855.85060973971;-0.0009 4.85358403645324e-10 2851.38773602932 3776.74979165462;-0.000825 4.9555472483567e-10 2957.01891334275 3694.6298975723;-0.00075 5.05354907161225e-10 3060.28629498077 3609.55657287959;-0.000675 5.14751116506184e-10 3161.10733057853 3521.59782389059;-0.0006 5.23735841684565e-10 3259.40142534279 3430.82396348342;-0.000525 5.3230190044453e-10 3355.09000447815 3337.30755489321;-0.00045 5.40442445209772e-10 3448.09657599852 3241.12335370614;-0.000375 5.4815096855336e-10 3538.34679187369 3142.34824810096;-0.0003 5.55421308399677e-10 3625.76850746195 3041.0611973858;-0.000225 5.62247652950291e-10 3710.29183918147 2937.34316887924;-0.00015 5.68624545329813e-10 3791.84922037412 2831.27707318633;-7.5e-05 5.74546887948047e-10 3870.37545531724 2722.94769792112]  x4=[-0.0015 -6.96769421526609e-11 1931.73943952997 4320.02713013533;-0.001425 -7.75649276830531e-11 2053.0969496025 4263.68907149476;-0.00135 -8.53909089970387e-11 2172.81324538696 4203.94268504708;-0.001275 -9.31486301248967e-11 2290.79262750821 4140.83573113945;-0.0012 -1.00831889663055e-10 2406.94078505334 4074.41865650526;-0.001125 -1.08434545731396e-10 2521.16487096232 4004.74455393775;-0.00105 -1.15950520882983e-10 2633.37357624857 3931.86911984848;-0.000975 -1.23373806962279e-10 2743.47720298994 3855.85060974441;-0.0009 -1.30698469907972e-10 2851.38773603184 3776.7497916594;-0.000825 -1.37918654496575e-10 2957.01891334526 3694.62989757715;-0.00075 -1.45028589022998e-10 3060.28629498325 3609.55657288451;-0.000675 -1.52022589914369e-10 3161.10733058099 3521.59782389557;-0.0006 -1.58895066273386e-10 3259.40142534522 3430.82396348847;-0.000525 -1.656405243476e-10 3355.09000448054 3337.30755489832;-0.00045 -1.72253571921035e-10 3448.09657600088 3241.1233537113;-0.000375 -1.78728922624645e-10 3538.34679187602 3142.34824810618;-0.0003 -1.85061400162153e-10 3625.76850746425 3041.06119739106;-0.000225 -1.91245942447905e-10 3710.29183918373 2937.34316888454;-0.00015 -1.97277605653426e-10 3791.84922037633 2831.27707319167;-7.5e-05 -2.03151568159436e-10 3870.37545531941 2722.94769792649]  x5=0.00142516474882927  V1=ones(3,3)  V2=ones(3,3)  I1=ones(3,3)  I2=ones(3,3)  nHarmo=1  Measurements=None  Decoupling=off  VsMag0=[ 1 1 1]  VrMag0=[ 1 1 1]  VsAngle0=[0 -120 120]  VrAngle0=[0 -120 120]  IsMag0=[ 1 1 1]  IrMag0=[ 1 1 1]  IsAngle0=[0 -120 120]  IrAngle0=[0 -120 120]
      settings: AttributesFormatString=\n  LibrarySourceBlock=sps_lib/Power Grid Elements/Distributed Parameters Line
  Decoupling_B : spsDistributedParametersLineLib/Distributed Parameters Line  Phases=3  Length=252  Frequency=60  Resistance="[0.01273  0.3864]/2"  Inductance="[0.9337e-3  4.1264e-3]/2"  Capacitance=[12.74e-9 7.751e-9]*2  x1=[-0.0015 1.28064071367027e-08 436042.69319822 659766.853671531;-0.001425 1.30154571680172e-08 454520.394369422 647175.964951811;-0.00135 1.32141028420148e-08 472634.758891759 634067.733667834;-0.001275 1.3402185364383e-08 490371.306419394 620452.638339124;-0.0012 1.35795543848313e-08 507715.858627609 606341.56266457;-0.001125 1.37460681172785e-08 524654.55054675 591745.786822158;-0.00105 1.39015934531946e-08 541173.841645668 576676.978451775;-0.000975 1.40460060680057e-08 557260.526655812 561147.183328271;-0.0009 1.41791905204772e-08 572901.746127319 545168.815732255;-0.000825 1.43010403449955e-08 588084.996708663 528754.648526305;-0.00075 1.44114581366752e-08 602798.14114164 511917.80294454;-0.000675 1.45103556292232e-08 617029.417963709 494671.738103706;-0.0006 1.45976537654971e-08 630767.450909925 477030.240244164;-0.000525 1.46732827607025e-08 644001.258006948 459007.411709378;-0.00045 1.47371821581777e-08 656720.260351871 440617.65967272;-0.000375 1.4789300877722e-08 668914.290568826 421875.684620596;-0.0003 1.48295972564287e-08 680573.600936631 402796.468601101;-0.000225 1.4858039081989e-08 691688.871180973 383395.263247599;-0.00015 1.48746036184427e-08 702251.215924888 363687.577586801;-7.5e-05 1.4879277624353e-08 712252.191791596 343689.165641087]  x2=[-0.0015 5.58282866623135e-09 437039.944981833 495282.668633326;-0.001425 5.76261547504192e-09 450867.190730282 482729.341007981;-0.00135 5.93779573721272e-09 464334.020144962 469790.12693344;-0.001275 6.10822941632251e-09 477429.668048486 456475.36981946;-0.0012 6.27378027029594e-09 490143.665980291 442795.713279153;-0.001125 6.43431596031335e-09 502465.850564961 428762.092620652;-0.00105 6.58970815660042e-09 514386.371636674 414385.72610559;-0.000975 6.73983264101302e-09 525895.700113277 399678.105981394;-0.0009 6.88456940633529e-09 536984.635613683 384650.989294556;-0.000825 7.02380275221158e-09 547644.31381252 369316.388492234;-0.00075 7.15742137763554e-09 557866.213526134 353686.561819681;-0.000675 7.28531846992244e-09 567642.163524295 337774.003521195;-0.0006 7.40739179009359e-09 576964.349062151 321591.43385241;-0.000525 7.52354375460463e-09 585825.318127217 305151.788911918;-0.00045 7.63368151335233e-09 594217.9873964 288468.210300348;-0.000375 7.73771702389749e-09 602135.647898298 271554.034615176;-0.0003 7.8355671218448e-09 609571.970376251 254422.782789648;-0.000225 7.92715358732309e-09 616521.010347849 237088.149284357;-0.00015 8.0124032075132e-09 622977.212856863 219563.991140099;-7.5e-05 8.0912478351731e-09 628935.41691379 201864.316900766]  x3=[-0.0015 2.4305719443952e-11 6141.18100421303 5250.26128906001;-0.001425 2.41053795388627e-11 6287.15453095554 5074.54796162879;-0.00135 2.38857701621946e-11 6428.1022025627 4894.77811820024;-0.001275 2.36470668663235e-11 6563.91134762239 4711.09546403662;-0.0012 2.33894604670116e-11 6694.47340238201 4523.64683224122;-0.001125 2.31131568908732e-11 6819.68399753263 4332.58206638224;-0.00105 2.28183770107594e-11 6939.4430416403 4138.05390071013;-0.000975 2.2505356469196e-11 7053.65480115751 3940.21783806414;-0.0009 2.21743454900147e-11 7162.22797695122 3739.23202556576;-0.000825 2.18256086783275e-11 7265.07577728592 3535.2571281983;-0.00075 2.14594248090059e-11 7362.11598720364 3328.45620037381;-0.000675 2.10760866038321e-11 7453.27103424534 3118.99455558983;-0.0006 2.06759004975022e-11 7538.46805046114 2907.03963428033;-0.000525 2.02591863926665e-11 7617.63893065983 2692.76086996639;-0.00045 1.98262774042044e-11 7690.72038685113 2476.32955381361;-0.000375 1.93775195929376e-11 7757.65399883715 2257.91869770463;-0.0003 1.89132716889943e-11 7818.38626091259 2037.70289593602;-0.000225 1.84339048050455e-11 7872.86862463638 1815.8581856503;-0.00015 1.79398021396437e-11 7921.05753764056 1592.56190611453;-7.5e-05 1.74313586708997e-11 7962.91447844539 1367.99255695803]  x4=[-0.0015 1.07143117341336e-11 -1150.93552720352 4266.75135249526;-0.001425 1.230875861012e-11 -1029.85223948753 4297.58364707668;-0.00135 1.38933660528038e-11 -907.945703648573 4324.98051904587;-0.001275 1.54668673512406e-11 -785.313369906152 4348.92006776255;-0.0012 1.70280046725678e-11 -662.053268671524 4369.38315631777;-0.001125 1.85755300674969e-11 -538.263932183675 4386.35342683163;-0.00105 2.01082064679053e-11 -414.044315744153 4399.81731352954;-0.000975 2.16248086757291e-11 -289.493718613716 4409.76405358648;-0.0009 2.31241243423682e-11 -164.711704634021 4416.18569573064;-0.000825 2.46049549378189e-11 -39.7980226378156 4419.07710659953;-0.00075 2.60661167087608e-11 85.1474732887566 4418.43597484356;-0.000675 2.75064416248307e-11 210.024903627982 4414.26281297363;-0.0006 2.89247783123283e-11 334.734443272735 4406.5609569515;-0.000525 3.0319992974607e-11 459.176401325145 4395.33656352302;-0.00045 3.16909702984133e-11 583.251300787971 4380.59860529657;-0.000375 3.30366143454511e-11 706.859958084991 4362.35886357045;-0.0003 3.43558494284584e-11 829.903562346837 4340.63191891512;-0.000225 3.56476209710946e-11 952.283754398894 4315.43513951771;-0.00015 3.69108963509534e-11 1073.90270538811 4286.78866729814;-7.5e-05 3.8144665725025e-11 1194.66319498591 4254.71540180799]  x5=0.00142516474882927  V1=ones(3,3)  V2=ones(3,3)  I1=ones(3,3)  I2=ones(3,3)  nHarmo=1  Measurements=None  Decoupling=off  VsMag0=[ 1 1 1]  VrMag0=[ 1 1 1]  VsAngle0=[0 -120 120]  VrAngle0=[0 -120 120]  IsMag0=[ 1 1 1]  IrMag0=[ 1 1 1]  IsAngle0=[0 -120 120]  IrAngle0=[0 -120 120]
      settings: AttributesFormatString=\n  LibrarySourceBlock=sps_lib/Power Grid Elements/Distributed Parameters Line
  Decoupling_C : spsDistributedParametersLineLib/Distributed Parameters Line  Phases=3  Length=252  Frequency=60  Resistance="[0.01273  0.3864]/2"  Inductance="[0.9337e-3  4.1264e-3]/2"  Capacitance=[12.74e-9 7.751e-9]*2  x1=[-0.0015 4.844801156156e-08 436042.693198114 659766.853671531;-0.001425 4.82512623993278e-08 454520.394369315 647175.964951808;-0.00135 4.80159419162025e-08 472634.758891653 634067.733667827;-0.001275 4.77422382237781e-08 490371.306419287 620452.638339114;-0.0012 4.74303701165982e-08 507715.858627502 606341.562664556;-0.001125 4.70805868972562e-08 524654.550546643 591745.786822141;-0.00105 4.66931681771056e-08 541173.841645561 576676.978451754;-0.000975 4.62684236527437e-08 557260.526655705 561147.183328247;-0.0009 4.58066928584444e-08 572901.746127213 545168.815732227;-0.000825 4.53083448947399e-08 588084.996708557 528754.648526273;-0.00075 4.47737781333676e-08 602798.141141534 511917.802944505;-0.000675 4.42034198988172e-08 617029.417963604 494671.738103668;-0.0006 4.35977261267346e-08 630767.45090982 477030.240244123;-0.000525 4.2957180999454e-08 644001.258006845 459007.411709333;-0.00045 4.22822965589493e-08 656720.260351768 440617.659672672;-0.000375 4.15736122975162e-08 668914.290568723 421875.684620545;-0.0003 4.083169472651e-08 680573.60093653 402796.468601047;-0.000225 4.00571369234854e-08 691688.871180873 383395.263247542;-0.00015 3.92505580580989e-08 702251.215924789 363687.577586741;-7.5e-05 3.84126028971544e-08 712252.191791498 343689.165641023]  x2=[-0.0015 1.96718210297772e-08 437039.944981809 495282.668633244;-0.001425 1.95315997315434e-08 450867.19073026 482729.341007901;-0.00135 1.93757651713276e-08 464334.020144941 469790.126933363;-0.001275 1.9204441920893e-08 477429.668048466 456475.369819384;-0.0012 1.90177669334246e-08 490143.665980273 442795.713279078;-0.001125 1.88158894340513e-08 502465.850564944 428762.09262058;-0.00105 1.85989708005571e-08 514386.371636659 414385.72610552;-0.000975 1.83671844343788e-08 525895.700113264 399678.105981326;-0.0009 1.8120715621991e-08 536984.635613671 384650.98929449;-0.000825 1.78597613867912e-08 547644.31381251 369316.38849217;-0.00075 1.75845303316023e-08 557866.213526126 353686.561819619;-0.000675 1.72952424719187e-08 567642.163524288 337774.003521136;-0.0006 1.69921290600291e-08 576964.349062146 321591.433852353;-0.000525 1.66754324001572e-08 585825.318127213 305151.788911863;-0.00045 1.63454056547673e-08 594217.987396398 288468.210300296;-0.000375 1.600231264219e-08 602135.647898298 271554.034615126;-0.0003 1.56464276257302e-08 609571.970376253 254422.782789601;-0.000225 1.52780350944248e-08 616521.010347853 237088.149284313;-0.00015 1.48974295356266e-08 622977.212856868 219563.991140057;-7.5e-05 1.4504915199596e-08 628935.416913797 201864.316900726]  x3=[-0.0015 8.26355596687612e-11 6141.18100421078 5250.26128905589;-0.001425 7.93421564659401e-11 6287.15453095334 5074.5479616246;-0.00135 7.59853283572158e-11 6428.10220256055 4894.77811819598;-0.001275 7.25677587396172e-11 6563.9113476203 4711.09546403229;-0.0012 6.90921795660062e-11 6694.47340237996 4523.64683223683;-0.001125 6.55613691611959e-11 6819.68399753065 4332.58206637779;-0.00105 6.19781500010007e-11 6939.44304163837 4138.05390070563;-0.000975 5.83453864559923e-11 7053.65480115564 3940.21783805958;-0.0009 5.46659825017652e-11 7162.22797694941 3739.23202556115;-0.000825 5.09428793975438e-11 7265.07577728417 3535.25712819365;-0.00075 4.71790533349842e-11 7362.11598720195 3328.45620036912;-0.000675 4.33775130590524e-11 7453.27103424372 3118.99455558511;-0.0006 3.95412974628793e-11 7538.46805045958 2907.03963427557;-0.000525 3.56734731585166e-11 7617.63893065834 2692.7608699616;-0.00045 3.17771320255334e-11 7690.72038684971 2476.3295538088;-0.000375 2.78553887394154e-11 7757.6539988358 2257.9186976998;-0.0003 2.39113782817408e-11 7818.38626091131 2037.70289593117;-0.000225 1.99482534341242e-11 7872.86862463516 1815.85818564543;-0.00015 1.59691822579308e-11 7921.05753763942 1592.56190610965;-7.5e-05 1.19773455617772e-11 7962.91447844432 1367.99255695314]  x4=[-0.0015 9.07056747959714e-11 -1150.93552720227 4266.75135249887;-0.001425 9.45400590214875e-11 -1029.85223948633 4297.58364708035;-0.00135 9.82988693703332e-11 -907.945703647417 4324.98051904959;-0.001275 1.01979101107027e-10 -785.313369905041 4348.92006776632;-0.0012 1.05577812310629e-10 -662.053268670461 4369.38315632158;-0.001125 1.09092126226465e-10 -538.26393218266 4386.35342683549;-0.00105 1.1251923356576e-10 -414.044315743187 4399.81731353344;-0.000975 1.15856394751345e-10 -289.493718612799 4409.76405359042;-0.0009 1.19100942107628e-10 -164.711704633154 4416.18569573461;-0.000825 1.22250281993096e-10 -39.7980226369996 4419.07710660354;-0.00075 1.25301896873631e-10 85.1474732895208 4418.43597484759;-0.000675 1.28253347334988e-10 210.024903628694 4414.26281297769;-0.0006 1.31102274032827e-10 334.734443273395 4406.56095695558;-0.000525 1.33846399578737e-10 459.176401325752 4395.33656352713;-0.00045 1.36483530360742e-10 583.251300788524 4380.59860530069;-0.000375 1.39011558296845e-10 706.859958085489 4362.35886357458;-0.0003 1.41428462520193e-10 829.903562347281 4340.63191891926;-0.000225 1.43732310994531e-10 952.283754399283 4315.43513952186;-0.00015 1.45921262058638e-10 1073.90270538845 4286.78866730229;-7.5e-05 1.47993565898525e-10 1194.66319498619 4254.71540181214]  x5=0.00142516474882927  V1=ones(3,3)  V2=ones(3,3)  I1=ones(3,3)  I2=ones(3,3)  nHarmo=1  Measurements=None  Decoupling=off  VsMag0=[ 1 1 1]  VrMag0=[ 1 1 1]  VsAngle0=[0 -120 120]  VrAngle0=[0 -120 120]  IsMag0=[ 1 1 1]  IrMag0=[ 1 1 1]  IsAngle0=[0 -120 120]  IrAngle0=[0 -120 120]
      settings: AttributesFormatString=\n  LibrarySourceBlock=sps_lib/Power Grid Elements/Distributed Parameters Line
  Load Flow Bus{,4,8,14} (4 alike) : spsLoadFlowBusLib/Load Flow Bus  LConnTagsString=a  Phases=single  Connectors=on one side  ID=MTL_13.8  Vbase=13.8e3  Vref=1  Vangle=0  VLF=1  VLFb=1  VLFc=1  angleLF=-47.86  angleLFb=0  angleLFc=0
      settings: AttributesFormatString=%<ID>\n%<Vbase>V\n%<VLF>pu\n%<angleLF>deg.
  Load Flow Bus{1,5,9,15} (4 alike) : spsLoadFlowBusLib/Load Flow Bus  LConnTagsString=a  Phases=single  Connectors=on one side  ID=MTL7  Vbase=735e3  Vref=1  Vangle=0  VLF=1.013  VLFb=1  VLFc=1  angleLF=-23.64  angleLFb=0  angleLFc=0
      settings: AttributesFormatString=%<ID>\n%<Vbase>V\n%<VLF>pu\n%<angleLF>deg.
  Load Flow Bus{2,6,10,12} (4 alike) : spsLoadFlowBusLib/Load Flow Bus  LConnTagsString=a  Phases=single  Connectors=on one side  ID=QUE7  Vbase=735e3  Vref=1  Vangle=0  VLF=1.023  VLFb=1  VLFc=1  angleLF=-14.99  angleLFb=0  angleLFc=0
      settings: AttributesFormatString=%<ID>\n%<Vbase>V\n%<VLF>pu\n%<angleLF>deg.
  Load Flow Bus{3,7,11,13} (4 alike) : spsLoadFlowBusLib/Load Flow Bus  LConnTagsString=a  Phases=single  Connectors=on one side  ID=SAG7  Vbase=735e3  Vref=1  Vangle=0  VLF=1.036  VLFb=1  VLFc=1  angleLF=-0.1653  angleLFb=0  angleLFc=0
      settings: AttributesFormatString=%<ID>\n%<Vbase>V\n%<VLF>pu\n%<angleLF>deg.
  MTL Load : Subsystem
  MTL Load1 : Subsystem
  MTL Load2 : Subsystem
  MTL Load3 : Subsystem
  MTL-QUE 5*219km : spsDistributedParametersLineLib/Distributed Parameters Line  Phases=3  Length=219  Frequency=60  Resistance="[0.01273  0.3864]/5"  Inductance="[0.9337e-3  4.1264e-3]/5"  Capacitance=[12.74e-9 7.751e-9]*5  x1=[-0.001275 1.10712408295317e-07 0 0;-0.0012 1.10111164476067e-07 0 0;-0.001125 1.09421899476692e-07 0 0;-0.00105 1.08645164285087e-07 0 0;-0.000975 1.07781579811479e-07 0 0;-0.0009 1.06831836392083e-07 0 0;-0.000825 1.05796693237257e-07 -131621.141335587 -623885.202244845;-0.00075 1.04676977824601e-07 -113930.944082935 -627356.84373319;-0.000675 1.03473585237484e-07 -96149.6721767847 -630326.985759538;-0.0006 1.02187477449527e-07 -78291.5396938359 -632793.254037795;-0.000525 1.00819682555617e-07 -60370.8221519566 -634753.677070836;-0.00045 9.93712939500652e-08 -42401.8450985535 -636206.687726483;-0.000375 9.78434694525616e-08 -24398.9726589487 -637151.124490251;-0.0003 9.62374303826328e-08 -6376.59605391708 -637586.23239384;-0.000225 9.45544605833383e-08 11650.8779044348 -637511.663618651;-0.00015 9.27959053949852e-08 29669.0383292544 -636927.47777382;-7.5e-05 9.09631705796843e-08 47663.481778785 -635834.141848573]  x2=[-0.001275 1.91780822359271e-08 0 0;-0.0012 1.89919571212853e-08 0 0;-0.001125 1.87906501267075e-08 0 0;-0.00105 1.85743221739249e-08 0 0;-0.000975 1.83431461921932e-08 0 0;-0.0009 1.8097306980055e-08 0 0;-0.000825 1.7837001057615e-08 -46015.2175618868 -658932.082245816;-0.00075 1.75624365094449e-08 -27368.4407499025 -659969.593736469;-0.000675 1.72738328182434e-08 -8699.7860251338 -660479.535631762;-0.0006 1.69714206893854e-08 9975.82317547212 -660461.500291947;-0.000525 1.66554418664999e-08 28643.4578556668 -659915.502134199;-0.00045 1.6326148938223e-08 47288.1953939113 -658841.97762109;-0.000375 1.59838051362834e-08 65895.1314722915 -657241.784911691;-0.0003 1.56286841250783e-08 84449.3919908021 -655116.203175571;-0.000225 1.52610697829104e-08 102936.144957474 -652466.931570246;-0.00015 1.48812559750603e-08 121340.612344843 -649296.087882902;-7.5e-05 1.44895463188746e-08 139648.081903277 -645606.206837468]  x3=[-0.001275 2.50723549709134e-10 0 0;-0.0012 2.17929357935265e-10 0 0;-0.001125 1.84960956767094e-10 0 0;-0.00105 1.5184470064008e-10 0 0;-0.000975 1.18607062182677e-10 0 0;-0.0009 8.5274611054514e-11 0 0;-0.000825 5.18739927070192e-11 -6146.00210112579 -16760.4201398047;-0.00075 1.84319070834531e-11 -5669.71860729473 -16927.4720622373;-0.000675 -1.5024912724618e-11 -5188.90282715859 -17080.9924225023;-0.0006 -4.84697218473458e-11 -4703.9391174953 -17220.8584987727;-0.000525 -8.18757850160404e-11 -4215.21515087417 -17346.9584842472;-0.00045 -1.15216397934935e-10 -3723.12160575638 -17459.1915765268;-0.000375 -1.4846490862819e-10 -3228.05185419262 -17557.4680581946;-0.0003 -1.81594738745077e-10 -2730.40164736747 -17641.709368535;-0.000225 -2.14579404806304e-10 -2230.56879924196 -17711.8481663334;-0.00015 -2.47392539374504e-10 -1728.95286854718 -17767.828383708;-7.5e-05 -2.8000791213196e-10 -1225.95483938316 -17809.6052709296]  x4=[-0.001275 5.99757540803851e-10 0 0;-0.0012 6.33068625330544e-10 0 0;-0.001125 6.65873644484422e-10 0 0;-0.00105 6.98146374435107e-10 0 0;-0.000975 7.29861016856067e-10 0 0;-0.0009 7.60992219547401e-10 0 0;-0.000825 7.91515096701999e-10 -488.21163409266 -6281.01987562245;-0.00075 8.21405248798881e-10 -310.448857287982 -6292.3115276641;-0.000675 8.50638782107795e-10 -132.437912416815 -6298.57320214612;-0.0006 8.79192327789502e-10 45.6789012951695 -6299.79989358175;-0.000525 9.07043060576467e-10 223.759199992369 -6295.99062137262;-0.00045 9.34168717019032e-10 401.660629008726 -6287.14843059266;-0.000375 9.60547613282473e-10 579.240976663867 -6273.28038955387;-0.0003 9.86158662480727e-10 756.358287944947 -6254.39758415609;-0.000225 1.01098139153293e-09 932.870977983314 -6230.51510902502;-0.00015 1.03499595752927e-09 1108.63794523529 -6201.65205544587;-7.5e-05 1.05818316359313e-09 1283.51868427656 -6167.83149610206]  x5=0.00123853603172068  V1=ones(3,3)  V2=ones(3,3)  I1=ones(3,3)  I2=ones(3,3)  nHarmo=1  Measurements=None  Decoupling=off  VsMag0=[ 1 1 1]  VrMag0=[ 1 1 1]  VsAngle0=[0 -120 120]  VrAngle0=[0 -120 120]  IsMag0=[ 1 1 1]  IrMag0=[ 1 1 1]  IsAngle0=[0 -120 120]  IrAngle0=[0 -120 120]
      settings: AttributesFormatString=\n  LibrarySourceBlock=sps_lib/Power Grid Elements/Distributed Parameters Line
  MTL-QUE 5*219km1 : spsDistributedParametersLineLib/Distributed Parameters Line  Phases=3  Length=219  Frequency=60  Resistance="[0.01273  0.3864]/5"  Inductance="[0.9337e-3  4.1264e-3]/5"  Capacitance=[12.74e-9 7.751e-9]*5  x1=[-0.001275 3.20321239875206e-08 0 0;-0.0012 3.32153156805333e-08 0 0;-0.001125 3.43719555584024e-08 0 0;-0.00105 3.55011190209066e-08 0 0;-0.000975 3.66019034320509e-08 0 0;-0.0009 3.76734288416195e-08 0 0;-0.000825 3.87148386885949e-08 -131621.141335636 -623885.202244844;-0.00075 3.97253004858795e-08 -113930.944082982 -627356.843733187;-0.000675 4.07040064857732e-08 -96149.6721768303 -630326.985759531;-0.0006 4.16501743256744e-08 -78291.5396938793 -632793.254037786;-0.000525 4.25630476534886e-08 -60370.8221519978 -634753.677070824;-0.00045 4.34418967322451e-08 -42401.8450985925 -636206.687726468;-0.000375 4.42860190234372e-08 -24398.9726589854 -637151.124490233;-0.0003 4.50947397486207e-08 -6376.59605395151 -637586.23239382;-0.000225 4.58674124288219e-08 11650.8779044027 -637511.663618627;-0.00015 4.66034194013224e-08 29669.0383292246 -636927.477773793;-7.5e-05 4.73021723134097e-08 47663.4817787576 -635834.141848544]  x2=[-0.001275 6.10205474030905e-09 0 0;-0.0012 6.26705307290048e-09 0 0;-0.001125 6.42704161915457e-09 0 0;-0.00105 6.58189248667534e-09 0 0;-0.000975 6.73148189004859e-09 0 0;-0.0009 6.87569024979407e-09 0 0;-0.000825 7.01440228795544e-09 -46015.2175619372 -658932.082245856;-0.00075 7.14750712025178e-09 -27368.4407499517 -659969.593736507;-0.000675 7.27489834471672e-09 -8699.78602518191 -660479.535631798;-0.0006 7.39647412675457e-09 9975.8231754252 -660461.50029198;-0.000525 7.51213728054534e-09 28643.4578556211 -659915.502134229;-0.00045 7.62179534673359e-09 47288.1953938668 -658841.977621118;-0.000375 7.72536066633905e-09 65895.1314722483 -657241.784911716;-0.0003 7.82275045082982e-09 84449.3919907603 -655116.203175593;-0.000225 7.91388684830229e-09 102936.144957434 -652466.931570265;-0.00015 7.99869700571475e-09 121340.612344804 -649296.087882919;-7.5e-05 8.07711312712502e-09 139648.08190324 -645606.206837482]  x3=[-0.001275 5.50526797346866e-10 0 0;-0.0012 5.4575319919563e-10 0 0;-0.001125 5.4054333428726e-10 0 0;-0.00105 5.34901367308051e-10 0 0;-0.000975 5.28831808360081e-10 0 0;-0.0009 5.22339509355907e-10 0 0;-0.000825 5.15429660140016e-10 -6146.00210112463 -16760.4201398041;-0.00075 5.08107784340147e-10 -5669.71860729353 -16927.4720622367;-0.000675 5.00379734951786e-10 -5188.90282715737 -17080.9924225018;-0.0006 4.92251689659372e-10 -4703.93911749405 -17220.8584987722;-0.000525 4.83730145897947e-10 -4215.21515087289 -17346.9584842467;-0.00045 4.74821915659211e-10 -3723.12160575508 -17459.1915765263;-0.000375 4.65534120046116e-10 -3228.05185419129 -17557.4680581942;-0.0003 4.55874183580367e-10 -2730.40164736612 -17641.7093685346;-0.000225 4.45849828267373e-10 -2230.56879924059 -17711.848166333;-0.00015 4.35469067423393e-10 -1728.95286854579 -17767.8283837077;-7.5e-05 4.24740199269814e-10 -1225.95483938174 -17809.6052709292]  x4=[-0.001275 -3.77375998653077e-10 0 0;-0.0012 -3.62747993460392e-10 0 0;-0.001125 -3.47830013071965e-10 0 0;-0.00105 -3.32633982693066e-10 0 0;-0.000975 -3.17172049797872e-10 0 0;-0.0009 -3.01456574418966e-10 0 0;-0.000825 -2.85500119266909e-10 -488.211634095954 -6281.01987562427;-0.00075 -2.69315439687808e-10 -310.448857291256 -6292.31152766579;-0.000675 -2.52915473466885e-10 -132.437912420065 -6298.57320214769;-0.0006 -2.3631333048621e-10 45.6789012919455 -6299.7998935832;-0.000525 -2.19522282244859e-10 223.759199989174 -6295.99062137395;-0.00045 -2.02555751249885e-10 401.660629005562 -6287.14843059386;-0.000375 -1.85427300286569e-10 579.240976660736 -6273.28038955494;-0.0003 -1.68150621576536e-10 756.358287941852 -6254.39758415703;-0.000225 -1.50739525832406e-10 932.870977980258 -6230.51510902584;-0.00015 -1.33207931217718e-10 1108.63794523227 -6201.65205544656;-7.5e-05 -1.15569852220964e-10 1283.51868427359 -6167.83149610262]  x5=0.00123853603172068  V1=ones(3,3)  V2=ones(3,3)  I1=ones(3,3)  I2=ones(3,3)  nHarmo=1  Measurements=None  Decoupling=off  VsMag0=[ 1 1 1]  VrMag0=[ 1 1 1]  VsAngle0=[0 -120 120]  VrAngle0=[0 -120 120]  IsMag0=[ 1 1 1]  IrMag0=[ 1 1 1]  IsAngle0=[0 -120 120]  IrAngle0=[0 -120 120]
      settings: AttributesFormatString=\n  LibrarySourceBlock=sps_lib/Power Grid Elements/Distributed Parameters Line
  MTL-QUE 5*219km2 : spsDistributedParametersLineLib/Distributed Parameters Line  Phases=3  Length=219  Frequency=60  Resistance="[0.01273  0.3864]/5"  Inductance="[0.9337e-3  4.1264e-3]/5"  Capacitance=[12.74e-9 7.751e-9]*5  x1=[-0.001275 1.33898360123561e-08 0 0;-0.0012 1.35660999900404e-08 0 0;-0.001125 1.37315194349609e-08 0 0;-0.00105 1.38859621133444e-08 0 0;-0.000975 1.40293045660769e-08 0 0;-0.0009 1.41614322073947e-08 0 0;-0.000825 1.42822394164832e-08 -163872.45963856 -773673.870997342;-0.00075 1.43916296219077e-08 -141934.751428668 -777997.405054968;-0.000675 1.44895153788118e-08 -119883.582750158 -781699.019890751;-0.0006 1.45758184388191e-08 -97736.5809698775 -784775.75649043;-0.000525 1.46504698125839e-08 -75511.4500621897 -787225.155357843;-0.00045 1.47134098249402e-08 -53225.9564566862 -789045.258481011;-0.000375 1.47645881626052e-08 -30897.9148359756 -790234.610897347;-0.0003 1.48039639143987e-08 -8545.17389489908 -790792.261856726;-0.000225 1.48315056039474e-08 13814.3979274434 -790717.765581505;-0.00015 1.48471912148459e-08 36162.9267314502 -790011.181622865;-7.5e-05 1.48510082082568e-08 58482.5474451391 -788673.074813212]  x2=[-0.001275 2.17886369034802e-09 0 0;-0.0012 2.20222585316057e-09 0 0;-0.001125 2.22382759032128e-09 0 0;-0.00105 2.24365163373199e-09 0 0;-0.000975 2.26168213635572e-09 0 0;-0.0009 2.27790468488455e-09 0 0;-0.000825 2.29230631126139e-09 -68511.7722423618 -808622.082896792;-0.00075 2.30487550304646e-09 -45624.1725038437 -810235.754253574;-0.000675 2.31560221262018e-09 -22700.1014998993 -811201.735545428;-0.0006 2.32447786521504e-09 242.115617860982 -811519.25458169;-0.000525 2.33149536577014e-09 23184.1391921008 -811188.0575425;-0.00045 2.33664910460293e-09 46107.6297201997 -810208.409181705;-0.000375 2.33993496189342e-09 68994.2625145706 -808581.092615214;-0.0003 2.34135031097759e-09 91825.742351135 -806307.408694992;-0.000225 2.34089402044701e-09 114583.818094245 -803389.174969176;-0.00015 2.33856645505338e-09 137250.297286361 -799828.724229156;-7.5e-05 2.33436947541683e-09 159807.060690827 -795628.902644778]  x3=[-0.001275 1.12323202915854e-10 0 0;-0.0012 1.09022399397285e-10 0 0;-0.001125 1.05634445040737e-10 0 0;-0.00105 1.02162048125085e-10 0 0;-0.000975 9.86079844312929e-11 0 0;-0.0009 9.49750950234995e-11 0 0;-0.000825 9.12662839779119e-11 -7102.47823834257 -20057.5471743786;-0.00075 8.74845160613334e-11 -6532.60058480674 -20250.3213202453;-0.000675 8.36328143611734e-11 -5957.50087031555 -20426.9076690889;-0.0006 7.9714257868838e-11 -5377.63882078146 -20587.165060484;-0.000525 7.57319790184314e-11 -4793.47796905466 -20730.965387124;-0.00045 7.16891611827356e-11 -4205.48528438208 -20858.1936972278;-0.000375 6.75890361284712e-11 -3614.13079911924 -20968.7482864312;-0.0003 6.34348814328726e-11 -3019.88723299364 -21062.540779087;-0.000225 5.92300178636429e-11 -2423.22961521982 -21139.4961989117;-0.00015 5.49778067243826e-11 -1824.63490476824 -21199.5530289201;-7.5e-05 5.06816471676155e-11 -1224.58160909164 -21242.6632606013]  x4=[-0.001275 -2.38943961746787e-11 0 0;-0.0012 -1.87062351349174e-11 0 0;-0.001125 -1.35031206170041e-11 0 0;-0.00105 -8.28921191107438e-12 0 0;-0.000975 -3.0686769359721e-12 0 0;-0.0009 2.15431109252047e-12 0 0;-0.000825 7.37557699768774e-12 -1323.85659522555 -8328.03394763995;-0.00075 1.25909469794532e-11 -1087.88942341655 -8362.13156092239;-0.000675 1.77962519508512e-11 -851.052609447738 -8389.54461417994;-0.0006 2.29873308707315e-11 -613.535477044478 -8410.25119383724;-0.000525 2.81600340700316e-11 -375.527893768275 -8424.23474737135;-0.00045 3.33102265689592e-11 -137.220119239563 -8431.48409654352;-0.000375 3.84337913824311e-11 101.19734695293 -8431.99344633495;-0.0003 4.35266328111286e-11 339.53391753464 -8425.76238957921;-0.000225 4.85846797155367e-11 577.599069897717 -8412.79590728772;-0.00015 5.36038887703507e-11 815.202498401879 -8393.10436466804;-7.5e-05 5.85802476966487e-11 1052.15426650184 -8366.70350283805]  x5=0.00123853603172068  V1=ones(3,3)  V2=ones(3,3)  I1=ones(3,3)  I2=ones(3,3)  nHarmo=1  Measurements=None  Decoupling=off  VsMag0=[ 1 1 1]  VrMag0=[ 1 1 1]  VsAngle0=[0 -120 120]  VrAngle0=[0 -120 120]  IsMag0=[ 1 1 1]  IrMag0=[ 1 1 1]  IsAngle0=[0 -120 120]  IrAngle0=[0 -120 120]
      settings: AttributesFormatString=\n  LibrarySourceBlock=sps_lib/Power Grid Elements/Distributed Parameters Line
  MTL-QUE 5*219km3 : spsDistributedParametersLineLib/Distributed Parameters Line  Phases=3  Length=219  Frequency=60  Resistance="[0.01273  0.3864]/5"  Inductance="[0.9337e-3  4.1264e-3]/5"  Capacitance=[12.74e-9 7.751e-9]*5  x1=[-0.001275 4.77489665600955e-08 0 0;-0.0012 4.74367309881795e-08 0 0;-0.001125 4.70865752193179e-08 0 0;-0.00105 4.66987791626746e-08 0 0;-0.000975 4.62736528164841e-08 0 0;-0.0009 4.58115360202426e-08 0 0;-0.000825 4.53127981830466e-08 -163872.459638586 -773673.870997235;-0.00075 4.47778379882921e-08 -141934.751428691 -777997.405054859;-0.000675 4.42070830749737e-08 -119883.582750177 -781699.019890641;-0.0006 4.36009896958362e-08 -97736.5809698939 -784775.756490319;-0.000525 4.29600423526533e-08 -75511.4500622029 -787225.155357731;-0.00045 4.22847534089244e-08 -53225.9564566961 -789045.258480898;-0.000375 4.15756626802989e-08 -30897.9148359823 -790234.610897233;-0.0003 4.08333370030557e-08 -8545.17389490259 -790792.261856611;-0.000225 4.00583697809833e-08 13814.3979274432 -790717.765581389;-0.00015 3.92513805110215e-08 36162.9267314532 -790011.181622749;-7.5e-05 3.84130142880455e-08 58482.5474451453 -788673.074813096]  x2=[-0.001275 7.13226982272139e-09 0 0;-0.0012 7.05593583860859e-09 0 0;-0.001125 6.97396144734584e-09 0 0;-0.00105 6.88641217800728e-09 0 0;-0.000975 6.79335801613925e-09 0 0;-0.0009 6.69487334781498e-09 0 0;-0.000825 6.59103690017147e-09 -68511.7722424217 -808622.082896655;-0.00075 6.48193167847621e-09 -45624.1725038994 -810235.754253435;-0.000675 6.36764489977405e-09 -22700.1014999507 -811201.735545287;-0.0006 6.24826792316725e-09 242.115617813834 -811519.254581546;-0.000525 6.12389617678437e-09 23184.139192058 -811188.057542354;-0.00045 5.99462908149653e-09 46107.6297201613 -810208.409181557;-0.000375 5.86056997144184e-09 68994.2625145366 -808581.092615064;-0.0003 5.7218260114217e-09 91825.7423511055 -806307.40869484;-0.000225 5.57850811123491e-09 114583.81809422 -803389.174969022;-0.00015 5.43073083701803e-09 137250.297286341 -799828.724229001;-7.5e-05 5.27861231966301e-09 159807.060690811 -795628.902644621]  x3=[-0.001275 8.18212190166438e-11 0 0;-0.0012 6.70674131271448e-11 0 0;-0.001125 5.22599945737577e-11 0 0;-0.00105 3.74108001803132e-11 0 0;-0.000975 2.25317001656089e-11 0 0;-0.0009 7.63458865453883e-12 0 0;-0.000825 -7.26862582988859e-12 -7102.47823834583 -20057.5471743794;-0.00075 -2.21660298860413e-11 -6532.60058481 -20250.321320246;-0.000675 -3.70457147570547e-11 -5957.50087031882 -20426.9076690895;-0.0006 -5.18957858505098e-11 -5377.63882078472 -20587.1650604846;-0.000525 -6.67043722467881e-11 -4793.47796905792 -20730.9653871244;-0.00045 -8.14596361885035e-11 -4205.48528438533 -20858.1936972282;-0.000375 -9.6149782543424e-11 -3614.13079912248 -20968.7482864315;-0.0003 -1.1076306823332e-10 -3019.88723299687 -21062.5407790872;-0.000225 -1.25287811621203e-10 -2423.22961522303 -21139.4961989118;-0.00015 -1.39712401849443e-10 -1824.63490477143 -21199.5530289201;-7.5e-05 -1.54025308121316e-10 -1224.58160909481 -21242.6632606012]  x4=[-0.001275 2.83833409601907e-10 0 0;-0.0012 2.983741627621e-10 0 0;-0.001125 3.12676400181858e-10 0 0;-0.00105 3.26728688871419e-10 0 0;-0.000975 3.40519795646214e-10 0 0;-0.0009 3.54038696106497e-10 0 0;-0.000825 3.67274583450086e-10 -1323.85659522454 -8328.03394763507;-0.00075 3.80216877111154e-10 -1087.88942341541 -8362.13156091751;-0.000675 3.92855231218173e-10 -851.052609446464 -8389.54461417506;-0.0006 4.05179542864243e-10 -613.535477043073 -8410.25119383237;-0.000525 4.17179960183202e-10 -375.527893766741 -8424.23474736649;-0.00045 4.28846890225058e-10 -137.2201192379 -8431.48409653868;-0.000375 4.40171006624446e-10 101.19734695472 -8431.99344633013;-0.0003 4.5114325705598e-10 339.533917536556 -8425.76238957441;-0.000225 4.61754870470547e-10 577.599069899757 -8412.79590728295;-0.00015 4.71997364106746e-10 815.202498404041 -8393.10436466331;-7.5e-05 4.8186255027188e-10 1052.15426650412 -8366.70350283335]  x5=0.00123853603172068  V1=ones(3,3)  V2=ones(3,3)  I1=ones(3,3)  I2=ones(3,3)  nHarmo=1  Measurements=None  Decoupling=off  VsMag0=[ 1 1 1]  VrMag0=[ 1 1 1]  VsAngle0=[0 -120 120]  VrAngle0=[0 -120 120]  IsMag0=[ 1 1 1]  IrMag0=[ 1 1 1]  IsAngle0=[0 -120 120]  IrAngle0=[0 -120 120]
      settings: AttributesFormatString=\n  LibrarySourceBlock=sps_lib/Power Grid Elements/Distributed Parameters Line
  MTL1 : spsThreePhaseVIMeasurementLib/Three-Phase V-I Measurement  VoltageMeasurement=phase-to-ground  SetLabelV=on  LabelV=Vabc_MTL7_1  Vpu=on  VpuLL=off  CurrentMeasurement=no  SetLabelI=off  LabelI=A1  Ipu=off  Pbase=100e6  Vbase=735e3  OutputType=Magnitude  PhasorSimulation=off  PSBequivalent=0
  MTL2 : spsThreePhaseVIMeasurementLib/Three-Phase V-I Measurement  VoltageMeasurement=phase-to-ground  SetLabelV=on  LabelV=Vabc_MTL7_2  Vpu=on  VpuLL=off  CurrentMeasurement=no  SetLabelI=off  LabelI=A1  Ipu=off  Pbase=100e6  Vbase=735e3  OutputType=Magnitude  PhasorSimulation=off  PSBequivalent=0
  MTL3 : spsThreePhaseVIMeasurementLib/Three-Phase V-I Measurement  VoltageMeasurement=phase-to-ground  SetLabelV=on  LabelV=Vabc_MTL7_4  Vpu=on  VpuLL=off  CurrentMeasurement=no  SetLabelI=off  LabelI=A1  Ipu=off  Pbase=100e6  Vbase=735e3  OutputType=Magnitude  PhasorSimulation=off  PSBequivalent=0
  MTL7 : spsThreePhaseVIMeasurementLib/Three-Phase V-I Measurement  VoltageMeasurement=phase-to-ground  SetLabelV=on  LabelV=Vabc_MTL7  Vpu=on  VpuLL=off  CurrentMeasurement=no  SetLabelI=off  LabelI=A1  Ipu=off  Pbase=100e6  Vbase=735e3  OutputType=Magnitude  PhasorSimulation=off  PSBequivalent=0
  North-West Network : Subsystem
  North-West Network1 : Subsystem
  North-West Network2 : Subsystem
  North-West Network3 : Subsystem
  North_East Network : Subsystem
  North_East Network1 : Subsystem
  North_East Network2 : Subsystem
  North_East Network3 : Subsystem
  PSS{,1..3} (4 alike) : Constant
  QUE Load and Wind Generation : Subsystem
  QUE Load and Wind Generation1 : Subsystem
  QUE Load and Wind Generation2 : Subsystem
  QUE Load and Wind Generation3 : Subsystem
  QUE{1..3,7} (4 alike) : spsThreePhaseVIMeasurementLib/Three-Phase V-I Measurement  VoltageMeasurement=no  SetLabelV=on  LabelV=Vabc_QUE7  Vpu=on  VpuLL=off  CurrentMeasurement=no  SetLabelI=off  LabelI=A1  Ipu=off  Pbase=100e6  Vbase=735e3  OutputType=Magnitude  PhasorSimulation=off  PSBequivalent=0
  Regulators1 : Subsystem
  Regulators2 : Subsystem
  Regulators3 : Subsystem
  Regulators5 : Subsystem
  SAG 660Mvar{,1..3} (4 alike) : spsThreePhaseSeriesRLCLoadLib/Three-Phase Series RLC Load  LConnTagsString=A|B|C  Configuration=Y (grounded)  NominalVoltage=735e3  Vabc=[1e3 1e3 1e3]  Vabcp=[1e3 1e3 1e3]  NominalFrequency=60  UnbalancedPower=off  ActivePower=2200000  InductivePower=660e6  CapacitivePower=0  Pabc=[10e3 9e3 11e3]  QLabc=[100 90 110]  QCabc=[100 90 110]  Pabcp=[10e3 9e3 11e3]  QLabcp=[100 90 110]  QCabcp=[100 90 110]  Measurements=None  LoadType=constant Z
  SAG-MIC 247km : spsDistributedParametersLineLib/Distributed Parameters Line  Phases=3  Length=247  Frequency=60  Resistance="[0.01273  0.3864]/1"  Inductance="[0.9337e-3  4.1264e-3]/1"  Capacitance=[12.74e-9 7.751e-9]*1  x1=[-0.001425 1.96878264857284e-08 -11926.9988578756 -635978.292860783;-0.00135 1.95671214240261e-08 6057.23046354862 -636061.280500396;-0.001275 1.94307747048444e-08 24036.6177276189 -635635.81048444;-0.0012 1.92788953216644e-08 41996.7904872504 -634702.222927138;-0.001125 1.91116046845413e-08 59923.3916551388 -633261.264124097;-0.00105 1.89290365230508e-08 77802.0909805967 -631314.085955738;-0.000975 1.87313367793877e-08 95618.5965049367 -628862.244966495;-0.0009 1.85186634917022e-08 113358.665986244 -625907.701120541;-0.000825 1.82911866677665e-08 131008.118284408 -622452.81623502;-0.00075 1.80490881490731e-08 148552.844697307 -618500.352092048;-0.000675 1.77925614654736e-08 165978.820239089 -614053.468230986;-0.0006 1.7521811680474e-08 183272.114851533 -609115.719422754;-0.000525 1.72370552273097e-08 200418.904539523 -603691.052828199;-0.00045 1.69385197359325e-08 217405.482421736 -597783.804842795;-0.000375 1.66264438510465e-08 234218.269687716 -591398.697630199;-0.0003 1.6301077041339e-08 250843.826452567 -584540.835347421;-0.000225 1.59626794000595e-08 267268.862500592 -577215.70006464;-0.00015 1.56115214371048e-08 283480.247909284 -569429.147382925;-7.5e-05 1.52478838627776e-08 299465.023545191 -561187.40175335]  x2=[-0.001425 6.78186914744446e-09 94383.5802767643 -641125.083483911;-0.00135 6.63574366783768e-09 112470.836606138 -638200.585428264;-0.001275 6.48431367627312e-09 130468.185469589 -634765.919589421;-0.0012 6.32770022356906e-09 148361.240061807 -630823.831586703;-0.001125 6.16602850412335e-09 166135.696948722 -626377.472664942;-0.00105 5.99942775583484e-09 183777.347501458 -621430.397175431;-0.000975 5.82803115679263e-09 201272.089254489 -615986.559734621;-0.0009 5.65197571881556e-09 218605.937178936 -610050.312062869;-0.000825 5.47140217792699e-09 235765.034861985 -603626.399505737;-0.00075 5.28645488185265e-09 252735.665583492 -596719.957240634;-0.000675 5.09728167463122e-09 269504.263280916 -589336.506171835;-0.0006 4.90403377843013e-09 286057.423393827 -581481.948517152;-0.000525 4.70686567266078e-09 302381.913579303 -573162.563089797;-0.00045 4.50593497049017e-09 318464.684289662 -564385.00027919;-0.000375 4.30140229284727e-09 334292.879204072 -555156.276734739;-0.0003 4.09343114002513e-09 349853.8455057 -545483.769756842;-0.000225 3.88218776098125e-09 365135.143996173 -535375.211399583;-0.00015 3.66784102044071e-09 380124.559039291 -524838.682289847;-7.5e-05 3.45056226390827e-09 394810.108326014 -513882.60516779]  x3=[-0.001425 2.28803124613519e-11 -438.079369964305 -3558.93637280654;-0.00135 2.20440623917546e-11 -337.290765732781 -3569.89847795688;-0.001275 2.11901906359669e-11 -236.232536423852 -3578.00686088522;-0.0012 2.03193797660055e-11 -134.985466439784 -3583.25503987431;-0.001125 1.94323258947561e-11 -33.6304911391919 -3585.63881961016;-0.00105 1.8529738119511e-11 67.7513678614534 -3585.15629453573;-0.000975 1.76123379551277e-11 169.079067455261 -3581.80785037418;-0.0009 1.66808587572609e-11 270.271607829542 -3575.59616382054;-0.000825 1.57360451361292e-11 371.248097215817 -3566.52620040199;-0.00075 1.47786523612852e-11 471.927816553465 -3554.60521050853;-0.000675 1.38094457578646e-11 572.230284015298 -3539.84272359706;-0.0006 1.28292000947968e-11 672.075319343505 -3522.25054057377;-0.000525 1.18386989654665e-11 771.383107944527 -3501.84272436058;-0.00045 1.08387341613214e-11 870.074264691616 -3478.63558865353;-0.000375 9.83010503892594e-12 968.069897384092 -3452.64768488181;-0.0003 8.81361788096801e-12 1065.29166981257 -3423.89978737809;-0.000225 7.79008525172891e-12 1161.6618643797 -3392.41487677175;-0.00015 6.76032534753187e-12 1257.10344422647 -3358.21812161862;-7.5e-05 5.72516134268847e-12 1351.54011481426 -3321.33685828152]  x4=[-0.001425 1.51093444642717e-11 -19.6739693555971 -1166.30624316245;-0.00135 1.58833394412689e-11 13.3057173491886 -1166.39655543667;-0.001275 1.664463751974e-11 46.2747676671099 -1165.55446815095;-0.0012 1.73926301296493e-11 79.2068266437857 -1163.78065445696;-0.001125 1.81267193371491e-11 112.075568895148 -1161.07653231425;-0.00105 1.88463183225589e-11 144.854719651548 -1157.44426335666;-0.000975 1.955085184946e-11 177.518075761411 -1152.88675116444;-0.0009 2.02397567245307e-11 210.039526637628 -1147.4076389431;-0.000825 2.09124822477545e-11 242.393075129963 -1141.01130661112;-0.00075 2.15684906526412e-11 274.552858306778 -1133.70286729868;-0.000675 2.2207257536109e-11 306.493168129462 -1125.48816326037;-0.0006 2.2828272277685e-11 338.188472003046 -1116.37376120489;-0.000525 2.34310384476864e-11 369.613433186568 -1106.36694704579;-0.00045 2.40150742040597e-11 400.742931046876 -1095.47572007721;-0.000375 2.45799126775572e-11 431.552081139677 -1083.70878657934;-0.0003 2.51251023449456e-11 462.016255101783 -1071.07555285878;-0.000225 2.56502073899463e-11 492.111100338647 -1057.58611772927;-0.00015 2.61548080516209e-11 521.812559491453 -1043.25126443885;-7.5e-05 2.6638500959921e-11 551.096889668201 -1028.08245204992]  x5=0.00139688767047948  V1=ones(3,3)  V2=ones(3,3)  I1=ones(3,3)  I2=ones(3,3)  nHarmo=1  Measurements=None  Decoupling=off  VsMag0=[ 1 1 1]  VrMag0=[ 1 1 1]  VsAngle0=[0 -120 120]  VrAngle0=[0 -120 120]  IsMag0=[ 1 1 1]  IrMag0=[ 1 1 1]  IsAngle0=[0 -120 120]  IrAngle0=[0 -120 120]
      settings: AttributesFormatString=\n  LibrarySourceBlock=sps_lib/Power Grid Elements/Distributed Parameters Line
  SAG-MIC 247km1 : spsDistributedParametersLineLib/Distributed Parameters Line  Phases=3  Length=247  Frequency=60  Resistance="[0.01273  0.3864]/1"  Inductance="[0.9337e-3  4.1264e-3]/1"  Capacitance=[12.74e-9 7.751e-9]*1  x1=[-0.001425 5.7304365423078e-09 -11926.9988579496 -635978.292860846;-0.00135 5.90796084327983e-09 6057.23046347575 -636061.280500456;-0.001275 6.08076241074858e-09 24036.6177275473 -635635.810484498;-0.0012 6.24870310978496e-09 41996.7904871801 -634702.222927192;-0.001125 6.41164869116374e-09 59923.3916550698 -633261.264124149;-0.00105 6.56946889868032e-09 77802.0909805291 -631314.085955786;-0.000975 6.72203757327554e-09 95618.5965048706 -628862.24496654;-0.0009 6.8692327538853e-09 113358.66598618 -625907.701120583;-0.000825 7.0109367749344e-09 131008.118284345 -622452.816235059;-0.00075 7.14703636039654e-09 148552.844697245 -618500.352092084;-0.000675 7.2774227143455e-09 165978.820239029 -614053.468231019;-0.0006 7.40199160792492e-09 183272.114851475 -609115.719422784;-0.000525 7.52064346266724e-09 200418.904539467 -603691.052828225;-0.00045 7.6332834300952e-09 217405.482421681 -597783.804842818;-0.000375 7.73982146754229e-09 234218.269687663 -591398.697630218;-0.0003 7.84017241013147e-09 250843.826452516 -584540.835347437;-0.000225 7.93425603885466e-09 267268.862500543 -577215.700064653;-0.00015 8.02199714469857e-09 283480.247909237 -569429.147382935;-7.5e-05 8.10332558876568e-09 299465.023545146 -561187.401753356]  x2=[-0.001425 2.12796509307411e-09 94383.5802766847 -641125.083483989;-0.00135 2.14187892597028e-09 112470.836606059 -638200.585428339;-0.001275 2.15408057362487e-09 130468.185469512 -634765.919589493;-0.0012 2.16456028222744e-09 148361.24006173 -630823.831586772;-0.001125 2.17330967445929e-09 166135.696948647 -626377.472665009;-0.00105 2.18032175619013e-09 183777.347501384 -621430.397175494;-0.000975 2.1855909220691e-09 201272.089254416 -615986.559734681;-0.0009 2.18911296000564e-09 218605.937178865 -610050.312062926;-0.000825 2.19088505453651e-09 235765.034861915 -603626.399505791;-0.00075 2.19090578907644e-09 252735.665583423 -596719.957240685;-0.000675 2.18917514705056e-09 269504.263280849 -589336.506171882;-0.0006 2.18569451190764e-09 286057.423393762 -581481.948517196;-0.000525 2.18046666601414e-09 302381.913579239 -573162.563089837;-0.00045 2.1734957884301e-09 318464.6842896 -564385.000279226;-0.000375 2.16478745156838e-09 334292.879204012 -555156.276734772;-0.0003 2.15434861674024e-09 349853.845505641 -545483.769756872;-0.000225 2.14218762859051e-09 365135.143996117 -535375.21139961;-0.00015 2.12831420842706e-09 380124.559039236 -524838.68228987;-7.5e-05 2.11273944644969e-09 394810.108325961 -513882.605167809]  x3=[-0.001425 1.66147796754637e-11 -438.079369964533 -3558.93637280684;-0.00135 1.65725573385204e-11 -337.290765733008 -3569.89847795718;-0.001275 1.65170871528092e-11 -236.232536424077 -3578.00686088551;-0.0012 1.6448413460348e-11 -134.985466440008 -3583.25503987459;-0.001125 1.63665911578357e-11 -33.6304911394141 -3585.63881961044;-0.00105 1.62716856527691e-11 67.7513678612331 -3585.15629453601;-0.000975 1.61637728111569e-11 169.079067455043 -3581.80785037445;-0.0009 1.60429388968734e-11 270.271607829326 -3575.5961638208;-0.000825 1.59092805027009e-11 371.248097215604 -3566.52620040225;-0.00075 1.57629044731148e-11 471.927816553254 -3554.60521050878;-0.000675 1.56039278188733e-11 572.230284015089 -3539.84272359731;-0.0006 1.54324776234816e-11 672.0753193433 -3522.25054057401;-0.000525 1.52486909416025e-11 771.383107944325 -3501.84272436081;-0.00045 1.50527146894974e-11 870.074264691416 -3478.63558865375;-0.000375 1.48447055275838e-11 968.069897383896 -3452.64768488203;-0.0003 1.46248297352031e-11 1065.29166981237 -3423.8997873783;-0.000225 1.43932630776995e-11 1161.66186437951 -3392.41487677196;-0.00015 1.41501906659159e-11 1257.10344422629 -3358.21812161881;-7.5e-05 1.38958068082191e-11 1351.54011481408 -3321.33685828171]  x4=[-0.001425 -9.78584724177595e-12 -19.673969355977 -1166.30624316279;-0.00135 -9.43513474786396e-12 13.3057173488131 -1166.396555437;-0.001275 -9.07687995159694e-12 46.2747676667389 -1165.55446815125;-0.0012 -8.71136923637754e-12 79.2068266434196 -1163.78065445725;-0.001125 -8.33889478587899e-12 112.075568894787 -1161.07653231452;-0.00105 -7.95975435047798e-12 144.854719651193 -1157.44426335692;-0.000975 -7.57425100923752e-12 177.518075761062 -1152.88675116469;-0.0009 -7.1826929276302e-12 210.039526637284 -1147.40763894333;-0.000825 -6.78539311119542e-12 242.393075129626 -1141.01130661133;-0.00075 -6.38266915532755e-12 274.552858306447 -1133.70286729888;-0.000675 -5.97484299139503e-12 306.493168129138 -1125.48816326055;-0.0006 -5.56224062939334e-12 338.188472002729 -1116.37376120506;-0.000525 -5.14519189733766e-12 369.613433186258 -1106.36694704594;-0.00045 -4.72403017760332e-12 400.742931046573 -1095.47572007735;-0.000375 -4.29909214042509e-12 431.552081139382 -1083.70878657946;-0.0003 -3.87071747476811e-12 462.016255101497 -1071.07555285888;-0.000225 -3.43924861678577e-12 492.111100338369 -1057.58611772935;-0.00015 -3.00503047608145e-12 521.812559491183 -1043.25126443892;-7.5e-05 -2.56841015999305e-12 551.09688966794 -1028.08245204997]  x5=0.00139688767047948  V1=ones(3,3)  V2=ones(3,3)  I1=ones(3,3)  I2=ones(3,3)  nHarmo=1  Measurements=None  Decoupling=off  VsMag0=[ 1 1 1]  VrMag0=[ 1 1 1]  VsAngle0=[0 -120 120]  VrAngle0=[0 -120 120]  IsMag0=[ 1 1 1]  IrMag0=[ 1 1 1]  IsAngle0=[0 -120 120]  IrAngle0=[0 -120 120]
      settings: AttributesFormatString=\n  LibrarySourceBlock=sps_lib/Power Grid Elements/Distributed Parameters Line
  SAG-MIC 247km2 : spsDistributedParametersLineLib/Distributed Parameters Line  Phases=3  Length=247  Frequency=60  Resistance="[0.01273  0.3864]/1"  Inductance="[0.9337e-3  4.1264e-3]/1"  Capacitance=[12.74e-9 7.751e-9]*1  x1=[-0.001425 2.31310520042732e-09 -89449.2345899237 -803563.355726914;-0.00135 2.3310203403533e-09 -66696.2840150374 -805770.954430128;-0.001275 2.347072098285e-09 -43890.0174511968 -807334.432161078;-0.0012 2.36124764269274e-09 -21048.6658789455 -808252.539099591;-0.001125 2.37353564186321e-09 1809.51167475409 -808524.541325025;-0.00105 2.38392627295789e-09 24666.2427325073 -808150.221402965;-0.000975 2.39241122986526e-09 47503.2559732264 -807129.878559028;-0.0009 2.3989837298406e-09 70302.2958379445 -805464.328439672;-0.000825 2.40363851892799e-09 93045.137123031 -803154.902460179;-0.00075 2.40637187616024e-09 115713.59954914 -800203.446740342;-0.000675 2.40718161653342e-09 138289.562294246 -796612.320628703;-0.0006 2.40606709275346e-09 160754.978479156 -792384.394816532;-0.000525 2.40302919575361e-09 183091.889593903 -787523.049043031;-0.00045 2.39807035398225e-09 205282.439853509 -782032.169393633;-0.000375 2.39119453146163e-09 227308.890471623 -775916.145193514;-0.0003 2.38240722461906e-09 249153.633840636 -769179.865498843;-0.000225 2.37171545789318e-09 270799.207606935 -761828.715188539;-0.00015 2.35912777811872e-09 292228.30863004 -753868.570659683;-7.5e-05 2.34465424769431e-09 313423.80681447 -745305.795130018]  x2=[-0.001425 1.09583173267483e-09 11099.4849220776 -821643.782394045;-0.00135 1.07553945054567e-09 34323.407660414 -821001.616626454;-0.001275 1.05438739863605e-09 57519.8927918324 -819703.154728278;-0.0012 1.03239248557263e-09 80670.3974010369 -817749.434670091;-0.001125 1.00957229375238e-09 103756.415328857 -815142.018225815;-0.00105 9.8594506528747e-10 126759.491965791 -811882.989724261;-0.000975 9.6152968742284e-10 149661.239004332 -807974.954382946;-0.0009 9.36345677437981e-10 172443.349138306 -803421.03622553;-0.000825 9.10413167045148e-10 195087.610697451 -798224.875584509;-0.00075 8.83752886296367e-10 217575.922205545 -792390.626191196;-0.000675 8.56386147012154e-10 239890.306850452 -785922.951855288;-0.0006 8.28334825745166e-10 262012.926854506 -778827.022736693;-0.000525 7.99621346292426e-10 283926.097733766 -771108.511212574;-0.00045 7.70268661770077e-10 305612.302434712 -762773.587342948;-0.000375 7.40300236265014e-10 327054.205337117 -753828.913938427;-0.0003 7.09740026078054e-10 348234.666111872 -744281.641234073;-0.000225 6.78612460573634e-10 369136.753422707 -734139.401173607;-0.00015 6.46942422651351e-10 389743.758460837 -723410.301308553;-7.5e-05 6.1475522885495e-10 410039.208301734 -712102.918317182]  x3=[-0.001425 4.96334857686293e-12 -974.267486516405 -4064.81506907863;-0.00135 4.92580706610975e-12 -858.96305833941 -4090.73328748314;-0.001275 4.88432794055529e-12 -742.971988236154 -4113.38143628795;-0.0012 4.83894435797788e-12 -626.386997693355 -4132.74141090944;-0.001125 4.78969259731904e-12 -509.301282968642 -4148.79773528012;-0.00105 4.73661202968265e-12 -391.808440590895 -4161.53757421994;-0.000975 4.67974508686233e-12 -274.002392540609 -4170.95074369659;-0.0009 4.61913722742207e-12 -155.977311170104 -4177.02971896642;-0.000825 4.55483690035737e-12 -37.8275439235824 -4179.7696405896;-0.00075 4.48689550636588e-12 80.3524620827707 -4179.16831831472;-0.000675 4.4153673567584e-12 198.468235560369 -4175.22623282959;-0.0006 4.34030963004331e-12 316.425356567126 -4167.94653537705;-0.000525 4.26178232621893e-12 434.129531985314 -4157.33504523584;-0.00045 4.17984821881043e-12 551.486670898037 -4143.40024506884;-0.000375 4.09457280468963e-12 668.402959804073 -4126.15327414207;-0.0003 4.00602425171782e-12 784.78493761095 -4105.60791942022;-0.000225 3.91427334425343e-12 900.539570346314 -4081.78060454549;-0.00015 3.81939342656802e-12 1015.57432552786 -4054.69037670882;-7.5e-05 3.7214603442161e-12 1129.79724613239 -4024.35889142386]  x4=[-0.001425 -9.04912567009818e-13 -279.355223169884 -1839.3774898859;-0.00135 -8.32188317345064e-13 -227.243591663481 -1846.54010495186;-0.001275 -7.58798829072332e-13 -174.950305106845 -1852.22662411095;-0.0012 -6.84802768625651e-13 -122.517165953136 -1856.43250164673;-0.001125 -6.10259287323565e-13 -69.9860884515402 -1859.15437544507;-0.00105 -5.35227974084472e-13 -17.399065141659 -1860.39006968169;-0.000975 -4.59768807792158e-13 35.201866714682 -1860.13859656153;-0.0009 -3.83942109349595e-13 87.7746587373776 -1858.40015710836;-0.000825 -3.07808493459329e-13 140.277285040876 -1855.17614100407;-0.00075 -2.31428820169019e-13 192.667775829027 -1850.46912547781;-0.000675 -1.54864146220845e-13 244.904250945097 -1844.28287324576;-0.0006 -7.81756762436837e-14 296.944953350121 -1836.62232950332;-0.000525 -1.42471382706115e-15 348.748282502847 -1827.49361797194;-0.00045 7.53273874839962e-14 400.272827614569 -1816.90403600394;-0.000375 1.52019273234046e-13 451.477400752275 -1804.86204874913;-0.0003 2.28589637103046e-13 502.321069763655 -1791.37728238786;-0.000225 3.04977269913684e-13 552.763190997637 -1776.46051643604;-0.00015 3.81121108561062e-13 602.763441794295 -1760.12367512813;-7.5e-05 4.56960284825605e-13 652.281852718173 -1742.37981788513]  x5=0.00139688767047948  V1=ones(3,3)  V2=ones(3,3)  I1=ones(3,3)  I2=ones(3,3)  nHarmo=1  Measurements=None  Decoupling=off  VsMag0=[ 1 1 1]  VrMag0=[ 1 1 1]  VsAngle0=[0 -120 120]  VrAngle0=[0 -120 120]  IsMag0=[ 1 1 1]  IrMag0=[ 1 1 1]  IsAngle0=[0 -120 120]  IrAngle0=[0 -120 120]
      settings: AttributesFormatString=\n  LibrarySourceBlock=sps_lib/Power Grid Elements/Distributed Parameters Line
  SAG-MIC 247km3 : spsDistributedParametersLineLib/Distributed Parameters Line  Phases=3  Length=247  Frequency=60  Resistance="[0.01273  0.3864]/1"  Inductance="[0.9337e-3  4.1264e-3]/1"  Capacitance=[12.74e-9 7.751e-9]*1  x1=[-0.001425 9.12227085445571e-09 -89449.2345900268 -803563.35572679;-0.00135 9.0586739694889e-09 -66696.2840151364 -805770.954429999;-0.001275 8.98783571915323e-09 -43890.0174512916 -807334.432160946;-0.0012 8.90981273046218e-09 -21048.6658790359 -808252.539099455;-0.001125 8.82466737379909e-09 1809.511674668 -808524.541324886;-0.00105 8.73246771305934e-09 24666.2427324257 -808150.221402822;-0.000975 8.63328745124099e-09 47503.2559731493 -807129.878558882;-0.0009 8.52720587152786e-09 70302.295837872 -805464.328439523;-0.000825 8.41430777391164e-09 93045.1371229631 -803154.902460028;-0.00075 8.2946834074042e-09 115713.599549077 -800203.446740187;-0.000675 8.16842839789378e-09 138289.562294188 -796612.320628546;-0.0006 8.03564367170323e-09 160754.978479103 -792384.394816372;-0.000525 7.89643537491099e-09 183091.889593855 -787523.049042869;-0.00045 7.75091478849957e-09 205282.439853465 -782032.169393468;-0.000375 7.59919823939919e-09 227308.890471584 -775916.145193348;-0.0003 7.44140700749786e-09 249153.633840602 -769179.865498675;-0.000225 7.27766722869209e-09 270799.207606906 -761828.715188369;-0.00015 7.10810979405574e-09 292228.308630016 -753868.570659511;-7.5e-05 6.93287024520775e-09 313423.806814451 -745305.795129844]  x2=[-0.001425 4.09175399971289e-09 11099.4849219547 -821643.782393909;-0.00135 3.99238398429015e-09 34323.4076602957 -821001.616626314;-0.001275 3.8898225181959e-09 57519.8927917188 -819703.154728134;-0.0012 3.78415158749688e-09 80670.3974009281 -817749.434669943;-0.001125 3.67545566391827e-09 103756.415328754 -815142.018225663;-0.00105 3.56382163731829e-09 126759.491965692 -811882.989724104;-0.000975 3.44933874622974e-09 149661.239004238 -807974.954382786;-0.0009 3.3320985065241e-09 172443.349138217 -803421.036225366;-0.000825 3.21219463825516e-09 195087.610697368 -798224.875584341;-0.00075 3.08972299074063e-09 217575.922205467 -792390.626191025;-0.000675 2.96478146594164e-09 239890.306850379 -785922.951855114;-0.0006 2.83746994020147e-09 262012.926854439 -778827.022736515;-0.000525 2.70789018440583e-09 283926.097733704 -771108.511212393;-0.00045 2.5761457826289e-09 305612.302434655 -762773.587342764;-0.000375 2.44234204932968e-09 327054.205337066 -753828.913938241;-0.0003 2.30658594516532e-09 348234.666111827 -744281.641233884;-0.000225 2.16898599148834e-09 369136.753422667 -734139.401173416;-0.00015 2.02965218359636e-09 389743.758460803 -723410.301308359;-7.5e-05 1.88869590280353e-09 410039.208301705 -712102.918316986]  x3=[-0.001425 1.30519196250036e-11 -974.267486517067 -4064.81506907854;-0.00135 1.26743073966411e-11 -858.963058340064 -4090.73328748303;-0.001275 1.22865635208692e-11 -742.9719882368 -4113.38143628782;-0.0012 1.18889979542095e-11 -626.386997693993 -4132.74141090929;-0.001125 1.14819285044929e-11 -509.301282969271 -4148.79773527994;-0.00105 1.10656805768092e-11 -391.808440591514 -4161.53757421974;-0.000975 1.0640586913383e-11 -274.002392541219 -4170.95074369638;-0.0009 1.02069873275847e-11 -155.977311170704 -4177.02971896619;-0.000825 9.76522843228883e-12 -37.8275439241713 -4179.76964058935;-0.00075 9.31566336279722e-12 80.3524620821931 -4179.16831831445;-0.000675 8.85865149454781e-12 198.468235559803 -4175.22623282931;-0.0006 8.39455815583559e-12 316.425356566572 -4167.94653537674;-0.000525 7.92375433577463e-12 434.129531984773 -4157.33504523552;-0.00045 7.44661638773516e-12 551.486670897509 -4143.40024506849;-0.000375 6.96352572849238e-12 668.402959803559 -4126.15327414171;-0.0003 6.47486853332777e-12 784.78493761045 -4105.60791941984;-0.000225 5.98103542732642e-12 900.539570345827 -4081.7806045451;-0.00015 5.48242117311738e-12 1015.57432552739 -4054.69037670841;-7.5e-05 4.97942435530641e-12 1129.79724613193 -4024.35889142343]  x4=[-0.001425 6.14953935760961e-12 -279.355223170233 -1839.37748988521;-0.00135 6.42583643009615e-12 -227.243591663809 -1846.54010495117;-0.001275 6.69699678725907e-12 -174.950305107152 -1852.22662411023;-0.0012 6.96280366765774e-12 -122.517165953421 -1856.43250164601;-0.001125 7.22304458933895e-12 -69.9860884518035 -1859.15437544433;-0.00105 7.47751151969173e-12 -17.3990651419001 -1860.39006968094;-0.000975 7.72600104174544e-12 35.201866714463 -1860.13859656077;-0.0009 7.96831451677815e-12 87.7746587371812 -1858.40015710759;-0.000825 8.20425824310546e-12 140.277285040702 -1855.17614100329;-0.00075 8.43364361092258e-12 192.667775828876 -1850.46912547701;-0.000675 8.65628725307621e-12 244.904250944968 -1844.28287324496;-0.0006 8.87201119164536e-12 296.944953350016 -1836.62232950251;-0.000525 9.08064298021423e-12 348.748282502765 -1827.49361797112;-0.00045 9.28201584172322e-12 400.27282761451 -1816.90403600312;-0.000375 9.47596880178794e-12 451.477400752239 -1804.8620487483;-0.0003 9.6623468173797e-12 502.321069763642 -1791.37728238702;-0.000225 9.84100090076451e-12 552.763190997647 -1776.46051643519;-0.00015 1.00117882386016e-11 602.763441794329 -1760.12367512729;-7.5e-05 1.01745723061063e-11 652.28185271823 -1742.37981788428]  x5=0.00139688767047948  V1=ones(3,3)  V2=ones(3,3)  I1=ones(3,3)  I2=ones(3,3)  nHarmo=1  Measurements=None  Decoupling=off  VsMag0=[ 1 1 1]  VrMag0=[ 1 1 1]  VsAngle0=[0 -120 120]  VrAngle0=[0 -120 120]  IsMag0=[ 1 1 1]  IrMag0=[ 1 1 1]  IsAngle0=[0 -120 120]  IrAngle0=[0 -120 120]
      settings: AttributesFormatString=\n  LibrarySourceBlock=sps_lib/Power Grid Elements/Distributed Parameters Line
  SAG{1..3,7} (4 alike) : spsThreePhaseVIMeasurementLib/Three-Phase V-I Measurement  VoltageMeasurement=no  SetLabelV=on  LabelV=Vabc_SAG7  Vpu=on  VpuLL=off  CurrentMeasurement=no  SetLabelI=off  LabelI=Iabc_SAG7  Ipu=off  Pbase=100e6  Vbase=735e3  OutputType=Magnitude  PhasorSimulation=off  PSBequivalent=0
  Subsystem : Subsystem
      mask Display: disp('Display\nWaveforms')
  Subsystem1 : Subsystem
      mask Display: disp('PSS_select')
  Subsystem2 : Subsystem
      mask Display: disp('Display\nWaveforms')
  Subsystem3 : Subsystem
      mask Display: disp('PSS_select')
  Subsystem4 : Subsystem
      mask Display: disp('Display\nWaveforms')
  Subsystem5 : Subsystem
      mask Display: disp('PSS_select')
  Subsystem6 : Subsystem
      mask Display: disp('Display\nWaveforms')
  Subsystem7 : Subsystem
      mask Display: disp('PSS_select')
  Three-Phase Fault{,1..3} (4 alike) : spsThreePhaseFaultLib/Three-Phase Fault  InitialStates=0  FaultA=on  FaultB=on  FaultC=on  GroundFault=on  SwitchTimes=[0.2 0.3]  External=off  SwitchStatus=NaN  FaultResistance=0.001  GroundResistance=0.001  SnubberResistance=1e6  SnubberCapacitance=inf  Measurements=None
  info : Subsystem
      settings: OpenFcn="showExample(\"simscapeelectricalsps/LoadFlow29BusNetworkExample\")"
      mask Display: disp('?')
  info1 : Subsystem
      settings: OpenFcn="showExample(\"simscapeelectricalsps/LoadFlow29BusNetworkExample\")"
      mask Display: disp('?')
  info2 : Subsystem
      settings: OpenFcn="showExample(\"simscapeelectricalsps/LoadFlow29BusNetworkExample\")"
      mask Display: disp('?')
  info3 : Subsystem
      settings: OpenFcn="showExample(\"simscapeelectricalsps/LoadFlow29BusNetworkExample\")"
      mask Display: disp('?')
  powergui{,1..3} (4 alike) : spspowerguiLib/powergui  Priority=1  SimulationMode=Discrete  SampleTime=75e-6  frequency=60  Iterations=50  frequencyindice=60  Pbase=1e+008  ErrMax=0.0001  UnitsV=kV  UnitsW=MW  buscounter=0  FunctionMessages=off  echomessages=off  EnableUseOfTLC=off  CurrentSourceSwitches=off  DisableSnubberDevices=off  DisableRonSwitches=off  DisableVfSwitches=off  DisplayEquations=off  AutomaticDiscreteSolvers=off  SolverType=Tustin/Backward Euler (TBE)  Interpol=off  ExternalGateDelay=off  methode=off  Ts=100  x0status=blocks  SPID=off  SwTol=0  HookPort=off  NonlinearTolerance=1e-4  nMaxIteration=100  ContinueOnMaxIteration=off  RestoreLinks=warning  ResistiveCurrentMeasurement=off  Frange=[0:2:500]  Ylog=off  Xlog=on  ShowGrid=off  save=off  variable=ZData  structure=0  ZoomFFT=off  StartTime=0.0  cycles=1  DisplayStyle=1  fundamental=60  FreqAxis=off  MaxFrequency=1000  frequencyindicesteady=1  RmsSteady=1  display=off
  wires:
  Regulators5/1(Pm) -> B_5 MTL-5000 MVA/1
  Regulators5/2(Vf) -> B_5 MTL-5000 MVA/2
  B_5 MTL-5000 MVA/1 -> Regulators5/1(m)
  PSS/1 -> Subsystem1/1(In1)
  B_5 MTL-5000 MVA1/1 -> Regulators1/1(m)
  PSS1/1 -> Subsystem3/1(In1)
  Regulators1/1(Pm) -> B_5 MTL-5000 MVA1/1
  Regulators1/2(Vf) -> B_5 MTL-5000 MVA1/2
  B_5 MTL-5000 MVA2/1 -> Regulators2/1(m)
  Regulators2/1(Pm) -> B_5 MTL-5000 MVA2/1
  Regulators2/2(Vf) -> B_5 MTL-5000 MVA2/2
  PSS2/1 -> Subsystem5/1(In1)
  Regulators3/2(Vf) -> B_5 MTL-5000 MVA3/2
  PSS3/1 -> Subsystem7/1(In1)
  B_5 MTL-5000 MVA3/1 -> Regulators3/1(m)
  Regulators3/1(Pm) -> B_5 MTL-5000 MVA3/1
  connections:
  QUE Load and Wind Generation/LConn3 -- Decoupling_C/RConn1 -- CHM-JCA 2*252km/RConn3 -- QUE7/LConn3 -- MTL-QUE 5*219km/RConn3 -- Load Flow Bus2/LConn1
  MTL7/RConn1 -- Three-Phase Fault/LConn1 -- MTL-QUE 5*219km/LConn1
  MTL7/RConn2 -- Three-Phase Fault/LConn2 -- MTL-QUE 5*219km/LConn2
  MTL7/RConn3 -- Three-Phase Fault/LConn3 -- MTL-QUE 5*219km/LConn3
  250 MW/LConn1 -- 5000 MVA 13.8 kV/735 kV1/LConn1 -- B_5 MTL-5000 MVA/RConn1
  250 MW/LConn2 -- 5000 MVA 13.8 kV/735 kV1/LConn2 -- B_5 MTL-5000 MVA/RConn2
  5000 MVA 13.8 kV/735 kV1/LConn3 -- Load Flow Bus/LConn1 -- 250 MW/LConn3 -- B_5 MTL-5000 MVA/RConn3
  MTL7/LConn3 -- MTL Load/LConn3 -- Decoupling_A/RConn1 -- North-West Network/RConn3 -- 5000 MVA 13.8 kV/735 kV1/RConn3 -- Load Flow Bus1/LConn1
  QUE Load and Wind Generation/LConn2 -- Decoupling_C/RConn2 -- CHM-JCA 2*252km/RConn2 -- QUE7/LConn2 -- MTL-QUE 5*219km/RConn2
  QUE Load and Wind Generation/LConn1 -- MTL-QUE 5*219km/RConn1 -- CHM-JCA 2*252km/RConn1 -- Decoupling_C/RConn3 -- QUE7/LConn1
  MTL7/LConn1 -- MTL Load/LConn1 -- Decoupling_A/RConn3 -- North-West Network/RConn1 -- 5000 MVA 13.8 kV/735 kV1/RConn1
  MTL7/LConn2 -- MTL Load/LConn2 -- Decoupling_A/RConn2 -- North-West Network/RConn2 -- 5000 MVA 13.8 kV/735 kV1/RConn2
  Cs SAG/LConn1 -- SAG7/RConn1 -- SAG 660Mvar/LConn1
  Cs SAG/LConn2 -- SAG7/RConn2 -- SAG 660Mvar/LConn2
  Cs SAG/LConn3 -- SAG7/RConn3 -- SAG 660Mvar/LConn3
  Load Flow Bus3/LConn1 -- CHM-SAG 117km/RConn3 -- SAG7/LConn3
  Cs CHMS/LConn1 -- CHM-SAG 117km/LConn1 -- North-West Network/RConn4
  Cs CHMS/LConn2 -- CHM-SAG 117km/LConn2 -- North-West Network/RConn5
  Cs CHMS/LConn3 -- CHM-SAG 117km/LConn3 -- North-West Network/RConn6
  Cs SAG/RConn1 -- SAG-MIC 247km/LConn1
  Cs SAG/RConn3 -- SAG-MIC 247km/LConn3
  Cs CHMS/RConn3 -- CHM-JCA 2*252km/LConn3
  Cs CHMS/RConn2 -- CHM-JCA 2*252km/LConn2
  Cs CHMS/RConn1 -- CHM-JCA 2*252km/LConn1
  Cs SAG/RConn2 -- SAG-MIC 247km/LConn2
  SAG7/LConn2 -- CHM-SAG 117km/RConn2
  SAG7/LConn1 -- CHM-SAG 117km/RConn1
  SAG-MIC 247km/RConn1 -- North_East Network/LConn1
  SAG-MIC 247km/RConn2 -- North_East Network/LConn2
  SAG-MIC 247km/RConn3 -- North_East Network/LConn3
  QUE7/RConn1 -- North_East Network/LConn4
  QUE7/RConn2 -- North_East Network/LConn5
  QUE7/RConn3 -- North_East Network/LConn6
  Load Flow Bus6/LConn1 -- MTL-QUE 5*219km1/RConn3 -- Decoupling_B/RConn1 -- QUE1/LConn3 -- CHM-JCA 2*252km1/RConn3 -- QUE Load and Wind Generation1/LConn3
  5000 MVA 13.8 kV/735 kV2/LConn3 -- 250 MW1/LConn3 -- B_5 MTL-5000 MVA1/RConn3 -- Load Flow Bus4/LConn1
  250 MW1/LConn2 -- 5000 MVA 13.8 kV/735 kV2/LConn2 -- B_5 MTL-5000 MVA1/RConn2
  5000 MVA 13.8 kV/735 kV2/RConn3 -- Decoupling_A/LConn1 -- North-West Network1/RConn3 -- MTL1/LConn3 -- MTL Load1/LConn3 -- Load Flow Bus5/LConn1
  MTL Load1/LConn1 -- MTL1/LConn1 -- Decoupling_A/LConn3 -- North-West Network1/RConn1 -- 5000 MVA 13.8 kV/735 kV2/RConn1
  CHM-SAG 117km1/LConn2 -- North-West Network1/RConn5 -- Cs CHMS1/LConn2
  MTL-QUE 5*219km1/LConn3 -- MTL1/RConn3 -- Three-Phase Fault1/LConn3
  MTL-QUE 5*219km1/RConn1 -- Decoupling_B/RConn3 -- QUE1/LConn1 -- CHM-JCA 2*252km1/RConn1 -- QUE Load and Wind Generation1/LConn1
  250 MW1/LConn1 -- 5000 MVA 13.8 kV/735 kV2/LConn1 -- B_5 MTL-5000 MVA1/RConn1
  5000 MVA 13.8 kV/735 kV2/RConn2 -- Decoupling_A/LConn2 -- North-West Network1/RConn2 -- MTL1/LConn2 -- MTL Load1/LConn2
  SAG1/RConn1 -- SAG 660Mvar1/LConn1 -- Cs SAG1/LConn1
  SAG1/RConn2 -- SAG 660Mvar1/LConn2 -- Cs SAG1/LConn2
  MTL-QUE 5*219km1/RConn2 -- Decoupling_B/RConn2 -- QUE1/LConn2 -- CHM-JCA 2*252km1/RConn2 -- QUE Load and Wind Generation1/LConn2
  CHM-SAG 117km1/RConn3 -- SAG1/LConn3 -- Load Flow Bus7/LConn1
  CHM-SAG 117km1/LConn3 -- North-West Network1/RConn6 -- Cs CHMS1/LConn3
  SAG1/RConn3 -- SAG 660Mvar1/LConn3 -- Cs SAG1/LConn3
  MTL-QUE 5*219km1/LConn1 -- MTL1/RConn1 -- Three-Phase Fault1/LConn1
  CHM-SAG 117km1/LConn1 -- North-West Network1/RConn4 -- Cs CHMS1/LConn1
  MTL-QUE 5*219km1/LConn2 -- MTL1/RConn2 -- Three-Phase Fault1/LConn2
  Cs CHMS1/RConn2 -- CHM-JCA 2*252km1/LConn2
  QUE1/RConn2 -- North_East Network1/LConn5
  Cs SAG1/RConn2 -- SAG-MIC 247km1/LConn2
  Cs SAG1/RConn3 -- SAG-MIC 247km1/LConn3
  Cs CHMS1/RConn1 -- CHM-JCA 2*252km1/LConn1
  SAG1/LConn2 -- CHM-SAG 117km1/RConn2
  SAG-MIC 247km1/RConn3 -- North_East Network1/LConn3
  SAG1/LConn1 -- CHM-SAG 117km1/RConn1
  QUE1/RConn3 -- North_East Network1/LConn6
  Cs CHMS1/RConn3 -- CHM-JCA 2*252km1/LConn3
  SAG-MIC 247km1/RConn2 -- North_East Network1/LConn2
  SAG-MIC 247km1/RConn1 -- North_East Network1/LConn1
  QUE1/RConn1 -- North_East Network1/LConn4
  Cs SAG1/RConn1 -- SAG-MIC 247km1/LConn1
  MTL-QUE 5*219km2/LConn1 -- MTL2/RConn1 -- Three-Phase Fault2/LConn1
  CHM-SAG 117km2/LConn3 -- North-West Network2/RConn6 -- Cs CHMS2/LConn3
  250 MW2/LConn1 -- 5000 MVA 13.8 kV/735 kV3/LConn1 -- B_5 MTL-5000 MVA2/RConn1
  MTL-QUE 5*219km2/LConn3 -- MTL2/RConn3 -- Three-Phase Fault2/LConn3
  5000 MVA 13.8 kV/735 kV3/LConn3 -- Load Flow Bus8/LConn1 -- 250 MW2/LConn3 -- B_5 MTL-5000 MVA2/RConn3
  CHM-SAG 117km2/RConn3 -- SAG2/LConn3 -- Load Flow Bus11/LConn1
  MTL-QUE 5*219km2/RConn1 -- QUE Load and Wind Generation2/LConn1 -- QUE2/LConn1 -- CHM-JCA 2*252km2/RConn1
  MTL Load2/LConn1 -- MTL2/LConn1 -- Decoupling_B/LConn3 -- North-West Network2/RConn1 -- 5000 MVA 13.8 kV/735 kV3/RConn1
  5000 MVA 13.8 kV/735 kV3/RConn2 -- Decoupling_B/LConn2 -- North-West Network2/RConn2 -- MTL2/LConn2 -- MTL Load2/LConn2
  5000 MVA 13.8 kV/735 kV3/RConn3 -- Decoupling_B/LConn1 -- North-West Network2/RConn3 -- MTL2/LConn3 -- MTL Load2/LConn3 -- Load Flow Bus9/LConn1
  Load Flow Bus10/LConn1 -- MTL-QUE 5*219km2/RConn3 -- QUE Load and Wind Generation2/LConn3 -- QUE2/LConn3 -- CHM-JCA 2*252km2/RConn3
  CHM-SAG 117km2/LConn2 -- North-West Network2/RConn5 -- Cs CHMS2/LConn2
  250 MW2/LConn2 -- 5000 MVA 13.8 kV/735 kV3/LConn2 -- B_5 MTL-5000 MVA2/RConn2
  SAG2/RConn3 -- SAG 660Mvar2/LConn3 -- Cs SAG2/LConn3
  MTL-QUE 5*219km2/RConn2 -- QUE Load and Wind Generation2/LConn2 -- QUE2/LConn2 -- CHM-JCA 2*252km2/RConn2
  MTL-QUE 5*219km2/LConn2 -- MTL2/RConn2 -- Three-Phase Fault2/LConn2
  CHM-SAG 117km2/LConn1 -- North-West Network2/RConn4 -- Cs CHMS2/LConn1
  SAG2/RConn1 -- SAG 660Mvar2/LConn1 -- Cs SAG2/LConn1
  SAG2/RConn2 -- SAG 660Mvar2/LConn2 -- Cs SAG2/LConn2
  Cs CHMS2/RConn2 -- CHM-JCA 2*252km2/LConn2
  SAG2/LConn1 -- CHM-SAG 117km2/RConn1
  Cs SAG2/RConn1 -- SAG-MIC 247km2/LConn1
  Cs SAG2/RConn3 -- SAG-MIC 247km2/LConn3
  QUE2/RConn3 -- North_East Network2/LConn6
  Cs CHMS2/RConn3 -- CHM-JCA 2*252km2/LConn3
  Cs CHMS2/RConn1 -- CHM-JCA 2*252km2/LConn1
  SAG-MIC 247km2/RConn1 -- North_East Network2/LConn1
  SAG-MIC 247km2/RConn3 -- North_East Network2/LConn3
  QUE2/RConn2 -- North_East Network2/LConn5
  SAG2/LConn2 -- CHM-SAG 117km2/RConn2
  Cs SAG2/RConn2 -- SAG-MIC 247km2/LConn2
  SAG-MIC 247km2/RConn2 -- North_East Network2/LConn2
  QUE2/RConn1 -- North_East Network2/LConn4
  MTL-QUE 5*219km3/LConn2 -- MTL3/RConn2 -- Three-Phase Fault3/LConn2
  CHM-JCA 2*252km3/RConn3 -- QUE3/LConn3 -- QUE Load and Wind Generation3/LConn3 -- MTL-QUE 5*219km3/RConn3 -- Load Flow Bus12/LConn1
  SAG3/RConn1 -- SAG 660Mvar3/LConn1 -- Cs SAG3/LConn1
  SAG3/RConn2 -- SAG 660Mvar3/LConn2 -- Cs SAG3/LConn2
  CHM-SAG 117km3/LConn2 -- North-West Network3/RConn5 -- Cs CHMS3/LConn2
  CHM-JCA 2*252km3/RConn2 -- QUE3/LConn2 -- QUE Load and Wind Generation3/LConn2 -- MTL-QUE 5*219km3/RConn2
  CHM-JCA 2*252km3/RConn1 -- QUE3/LConn1 -- QUE Load and Wind Generation3/LConn1 -- MTL-QUE 5*219km3/RConn1
  CHM-SAG 117km3/LConn1 -- North-West Network3/RConn4 -- Cs CHMS3/LConn1
  North-West Network3/RConn2 -- Decoupling_C/LConn2 -- 5000 MVA 13.8 kV/735 kV4/RConn2 -- MTL3/LConn2 -- MTL Load3/LConn2
  5000 MVA 13.8 kV/735 kV4/RConn3 -- North-West Network3/RConn3 -- Decoupling_C/LConn1 -- MTL3/LConn3 -- MTL Load3/LConn3 -- Load Flow Bus15/LConn1
  250 MW3/LConn1 -- 5000 MVA 13.8 kV/735 kV4/LConn1 -- B_5 MTL-5000 MVA3/RConn1
  MTL-QUE 5*219km3/LConn1 -- MTL3/RConn1 -- Three-Phase Fault3/LConn1
  5000 MVA 13.8 kV/735 kV4/LConn3 -- Load Flow Bus14/LConn1 -- 250 MW3/LConn3 -- B_5 MTL-5000 MVA3/RConn3
  MTL Load3/LConn1 -- MTL3/LConn1 -- North-West Network3/RConn1 -- Decoupling_C/LConn3 -- 5000 MVA 13.8 kV/735 kV4/RConn1
  MTL-QUE 5*219km3/LConn3 -- MTL3/RConn3 -- Three-Phase Fault3/LConn3
  CHM-SAG 117km3/RConn3 -- SAG3/LConn3 -- Load Flow Bus13/LConn1
  CHM-SAG 117km3/LConn3 -- North-West Network3/RConn6 -- Cs CHMS3/LConn3
  SAG3/RConn3 -- SAG 660Mvar3/LConn3 -- Cs SAG3/LConn3
  250 MW3/LConn2 -- 5000 MVA 13.8 kV/735 kV4/LConn2 -- B_5 MTL-5000 MVA3/RConn2
  QUE3/RConn3 -- North_East Network3/LConn6
  SAG-MIC 247km3/RConn2 -- North_East Network3/LConn2
  SAG3/LConn1 -- CHM-SAG 117km3/RConn1
  QUE3/RConn1 -- North_East Network3/LConn4
  SAG-MIC 247km3/RConn3 -- North_East Network3/LConn3
  SAG3/LConn2 -- CHM-SAG 117km3/RConn2
  SAG-MIC 247km3/RConn1 -- North_East Network3/LConn1
  QUE3/RConn2 -- North_East Network3/LConn5
  Cs SAG3/RConn1 -- SAG-MIC 247km3/LConn1
  Cs CHMS3/RConn2 -- CHM-JCA 2*252km3/LConn2
  Cs SAG3/RConn2 -- SAG-MIC 247km3/LConn2
  Cs CHMS3/RConn1 -- CHM-JCA 2*252km3/LConn1
  Cs CHMS3/RConn3 -- CHM-JCA 2*252km3/LConn3
  Cs SAG3/RConn3 -- SAG-MIC 247km3/LConn3
